simulink library "did"  (R2021b)
settings: Solver=VariableStepAuto  StartTime=0.0  StopTime=10.0  RelTol=1e-3
undefined symbols (not defined in the file or in its folder): ADID_DODRange_pct, ADID_SOCRange_pct, ADID_TempRange_C, DiscIntNeverNeededParam, ENUM_CHRGPLUGSTA_AC, ENUM_CHRGPLUGSTA_DC, ENUM_CHRGPLUGSTA_NONE, ENUM_DRIVETRAIN_AWD, ENUM_DRIVETRAIN_FWD, ENUM_DRIVETRAIN_RWD, ENUM_EXTCHRGSTS_CHARGING, ENUM_OBCV2LSTA_WORKING, ENUM_PWRSTASW_READY, ENUM_VEHICLETYPE_D31HAWD, ENUM_VEHICLETYPE_D31HRWD, HOUR2SEC, HUNDRED, KDID_CPSAVehSpdThres_kph, KDID_DIDModelVersion_raw, KDID_DoDChrgCycle_s, KDID_FiveKmEquivEnergy_Wh, KDID_FlashInitDIDModelVersion_raw, KDID_IPSAVehSpdThres_kph, KDID_PropActiveTripThres_s, KDID_PSARResetThres_sec, KDID_RESSCNTSDODRNGAXIS_enum, KDID_RESSTIMESOCRNGAXIS_enum, KDID_RESSTTEMPRNGAXIS_enum, KDID_WarnUpPropActiveThres_s, KDID_WarnUpVehOperIdleThres_mph, KDID_WarnUpVehOperIdleThres_s, KDID_WarnUpVehOperThres_mph, KDID_WarnUpVehOperThres_s, KPH2MPH, KXX2XX, MINUSONE_FLOAT, ONE_FLOAT, ONE_INT, ONE_INT16, ONE_PERCENT, TRUE, UINT16_MAX, UINT32_MAX, XX2KXX, ZERO_FLOAT, ZERO_INT, ZERO_INT16, ZERO_INT32
libraries: hcu_lib x112, simulink x10, nmm x1
(part 2 of 4)

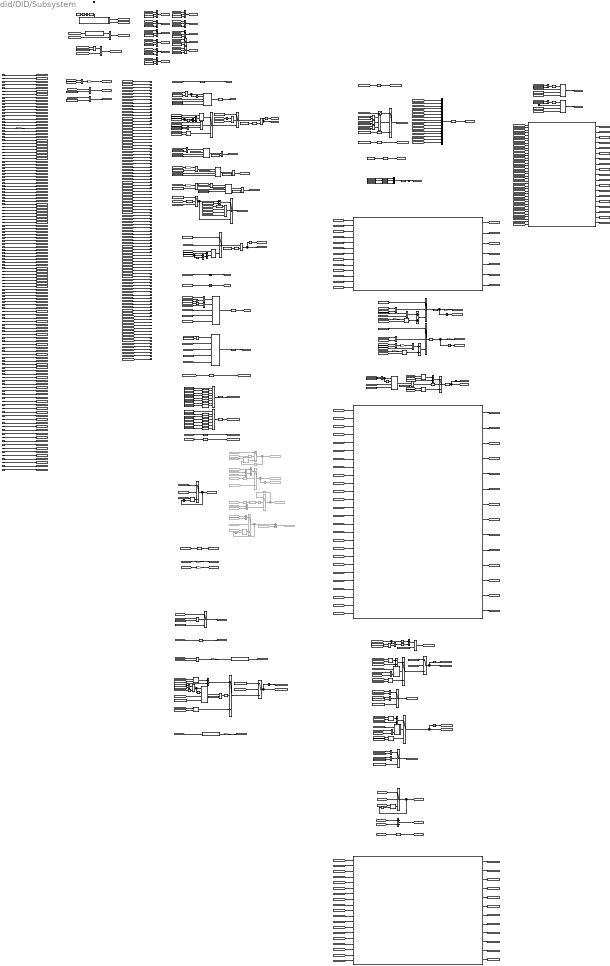
== system did/DID/Subsystem ==
  note: Flash data selector
  note: Model Version
  note: 0xF810: Protocol Identification
  note: 0xF896: Total Number of Propulsion System Active Events
  note: code_clear ??
  note: 0xF44D: Engine run time while MIL activated
  note: 0xF431: Distance traveled since DTCs cleared
  note: 0xF430: Number of warm-ups since DTCs cleared
  note: add debounce?
  note: 0xF421: Distance Traveled While MIL is Activated
  note: 0xF41F: Time Since Engine Start
  note: 0xF40D: Vehicle Speed Sensor
  note: 0xF449: Accelerator Pedal Position D
  note: 0xF44A: Accelerator Pedal Position E
  note: add debounce?
  note: 0xF44E: Engine run time since DTCs cleared
  note: 0xF45B: Hybrid Battery Pack Remaining Charge
  note: 0xF49A: Hybrid/EV Battery System Voltage
  note: 0xF4D1
  note: 0xF4DA
  note: 0xF4D4
  note: 0xF4B9
  note: 0xF4D6
  note: 0xF4D0
  note: SOH?
  note: 0xF4A6
  note: 0xF4B2
  note: Annex G
  note: Annex B
  note: 0xF802: Vehicle Identification Number
  note: 0xF804: Calibration Identifications
  note: 0xF813: Certification Test Group/Engine Family Number
  note: 0xF80A: ECUNAME
  note: 0xF881: High Voltage Battery Net Amp Hours
  note: 0xF882: Ignition Counter
  note: 0xF88C: Positive Kinetic Energy
  note: 0xF88D: Total Distance Travelled
  task_time_s : Inport
  VTQD_VehActSpd_kph : Inport  Port=2
  VPMM_SysPowerMode_enum : Inport  Port=3
  VPMM_DrivetrainSelect_enum : Inport  Port=4
  VDDM_VehMalfunLevel_enum : Inport  Port=5
  VDDM_LimpHomeActTmp_flg : Inport  Port=6
  VDDM_EnterNewOperCyc_flg : Inport  Port=7
  VINP_CANMsgValidESC1_flg : Inport  Port=8
  VINP_ODOMETER_km : Inport  Port=9
  VINP_CANMsgValidMETER1_flg : Inport  Port=10
  VINP_ClearDTCcmd_flg : Inport  Port=11
  VDHP_LowIdleAccPedal_flg : Inport  Port=12
  VDHP_EAPS1NRM_pct : Inport  Port=13
  VDHP_EAPS2NRM_pct : Inport  Port=14
  VINP_HVBattSOC_pct : Inport  Port=15
  VINP_HVBattPackVolt_V : Inport  Port=16
  VINP_ExtChrgSta_enum : Inport  Port=17
  VINP_HVBattCurr_A : Inport  Port=18
  VINP_HVBattVolt_V : Inport  Port=19
  VINP_ChrgPlugSta_enum : Inport  Port=20
  VINP_HVBPwrAvailChrg_kW : Inport  Port=21
  VINP_HVBCellVoltMax_mV : Inport  Port=22
  VINP_HVBCellVoltMin_mV : Inport  Port=23
  VINP_HVBSOH_pct : Inport  Port=24
  VINP_CANMsgValidMCUBR1_flg : Inport  Port=25
  VINP_CANMsgValidBMS6_flg : Inport  Port=26
  VINP_CANMsgValidBMS1_flg : Inport  Port=27
  VINP_CANMsgValidCCU2_flg : Inport  Port=28
  VINP_CANMsgValidBMS4_flg : Inport  Port=29
  VINP_CellTempAvg_C : Inport  Port=30
  VINP_OBCV2LSta_enum : Inport  Port=31
  VINP_RrMCUDCBusCurr_A : Inport  Port=32
  VINP_RrMCUDCBusVolt_V : Inport  Port=33
  VINP_FrMCUDCBusCurr_A : Inport  Port=34
  VINP_FrMCUDCBusVolt_V : Inport  Port=35
  VINP_CANMsgValidMCUBF1_flg : Inport  Port=36
  VINP_HVBMTempMax_C : Inport  Port=37
  VINP_HVBMTempMin_C : Inport  Port=38
  VINP_MCUBRRealPwrKwSta_kW : Inport  Port=39
  VINP_MCUBFRealPwrKwSta_kW : Inport  Port=40
  VINP_CANMsgValidBMS3_flg : Inport  Port=41
  VINP_VehicleType_enum : Inport  Port=42
  VINP_CarModel1_cnt : Inport  Port=43
  VINP_CarModel2_cnt : Inport  Port=44
  VINP_CarModel3_cnt : Inport  Port=45
  VINP_ECU1_cnt : Inport  Port=46
  VINP_ECU2_cnt : Inport  Port=47
  VINP_Major1_cnt : Inport  Port=48
  VINP_Major2_cnt : Inport  Port=49
  VINP_Minor1_cnt : Inport  Port=50
  VINP_Minor2_cnt : Inport  Port=51
  VINP_Patch1_cnt : Inport  Port=52
  VINP_Patch2_cnt : Inport  Port=53
  VINP_Country1_cnt : Inport  Port=54
  VINP_Country2_cnt : Inport  Port=55
  VINP_Variation_cnt : Inport  Port=56
  VINP_ECUGen1_cnt : Inport  Port=57
  VINP_ECUGen2_cnt : Inport  Port=58
  VINP_FlashMILDIST_km : Inport  Port=59
  VINP_FlashWARMUPS_cnt : Inport  Port=60
  VINP_FlashDelayCLRDIST_km : Inport  Port=61
  VINP_FlashMILTime_min : Inport  Port=62
  VINP_FlashCLRTime_min : Inport  Port=63
  VINP_FlashNUMPSATRIPSFLTMEMCLR_cnt : Inport  Port=64
  VINP_FlashPSAR_sec : Inport  Port=65
  VINP_FlashPSAL_sec : Inport  Port=66
  VINP_FlashIPSAR_sec : Inport  Port=67
  VINP_FlashIPSAL_sec : Inport  Port=68
  VINP_FlashCPSAR_sec : Inport  Port=69
  VINP_FlashCPSAL_sec : Inport  Port=70
  VINP_FlashHVBNAH_Ah : Inport  Port=71
  VINP_FlashIGNCNTR_cnt : Inport  Port=72
  VINP_FlashTNBCPSAR_Ahr : Inport  Port=73
  VINP_FlashTNBCPSAL_Ahr : Inport  Port=74
  VINP_FlashTNECPSAR_kWh : Inport  Port=75
  VINP_FlashTNECPSAL_kWh : Inport  Port=76
  VINP_FlashTEBPSAR_kWh : Inport  Port=77
  VINP_FlashTEBPSAL_kWh : Inport  Port=78
  VINP_FlashTGEOVCR_kWh : Inport  Port=79
  VINP_FlashTGEOVCL_kWh : Inport  Port=80
  VINP_FlashGECHGOVCDCR_kWh : Inport  Port=81
  VINP_FlashGECHGOVCDCL_kWh : Inport  Port=82
  VINP_FlashGECHGOVCACR_kWh : Inport  Port=83
  VINP_FlashGECHGOVCACL_kWh : Inport  Port=84
  VINP_FlashRESSV2XENNONPSAR_kWh : Inport  Port=85
  VINP_FlashRESSV2XENNONPSAL_kWh : Inport  Port=86
  VINP_FlashODOMETER_km : Inport  Port=87
  VINP_FlashPKERNumerator_kphsqr : Inport  Port=88
  VINP_FlashPKELNumerator_kphsqr : Inport  Port=89
  VINP_FlashResetCDEODTR_km : Inport  Port=90
  VINP_FlashTempPSAR_sec : Inport  Port=91
  VINP_FlashAvgBattTempPSAR_C : Inport  Port=92
  VINP_FlashTempPSAL_sec : Inport  Port=93
  VINP_FlashAvgBattTempPSAL_C : Inport  Port=94
  VINP_FlashOVCR_sec : Inport  Port=95
  VINP_FlashAvgBattTempOVCR_C : Inport  Port=96
  VINP_FlashOVCL_sec : Inport  Port=97
  VINP_FlashAvgBattTempOVCL_C : Inport  Port=98
  VINP_FlashOFFR_sec : Inport  Port=99
  VINP_FlashAvgBattTempOFFR_C : Inport  Port=100
  VINP_FlashOFFL_sec : Inport  Port=101
  VINP_FlashAvgBattTempOFFL_C : Inport  Port=102
  VINP_FlashHVBNE_kWh : Inport  Port=103
  VINP_FlashQTYPSATRIPSR_cnt : Inport  Port=104
  VINP_FlashQTYPSATRIPSL_cnt : Inport  Port=105
  VINP_FlashRESSCNTDODRNGR_cnt : Inport  Port=106
  VINP_FlashETMBTOER_kWh : Inport  Port=107
  VINP_FlashETMBTOEL_kWh : Inport  Port=108
  VINP_FlashRESSCNTDODRNGL_cnt : Inport  Port=109
  VINP_FlashETMATOER_kWh : Inport  Port=110
  VINP_FlashETMATOEL_kWh : Inport  Port=111
  VINP_FlashRESSTIMESOCPSARNGR_s : Inport  Port=112
  VINP_FlashRESSTIMESOCPSARNGL_s : Inport  Port=113
  VINP_FlashRESSTIMESOCCHGRNGR_s : Inport  Port=114
  VINP_FlashRESSTIMESOCOFFRNGL_s : Inport  Port=115
  VINP_FlashMAXBATTEMPL_C : Inport  Port=116
  VINP_FlashMINBATTEMPL_C : Inport  Port=117
  VINP_FlashRESSTIMESOCCHGRNGL_s : Inport  Port=118
  VINP_FlashRESSTIMESOCOFFRNGR_s : Inport  Port=119
  VINP_FlashAVGBATTEMPL_sec : Inport  Port=120
  VINP_FlashAVGBATTEMPL_C : Inport  Port=121
  VINP_VinCode_cnt : Inport  Port=122
  VINP_FlashModelVersion_raw : Inport  Port=123
  VINP_FlashModelVersionChksum_raw : Inport  Port=124
  Enable : EnablePort
  0xF819: Total Propulsion System Active Time : Subsystem
  0xF885 - 0xF88B : Subsystem
  0xF88E - 0xF890 : Subsystem
  0xF898-0xF8 : Subsystem
  1-D Lookup Table : Lookup_n-D  NumberOfTableDimensions=1  BreakpointsForDimension1=[ENUM_DRIVETRAIN_RWD;ENUM_DRIVETRAIN_FWD;ENUM_DRIVETRAIN_AWD]  Table=[uint8('R');uint8('F');uint8('A')]  InterpMethod=Nearest  InternalRulePriority=Speed  RndMeth=Simplest  InputSameDT=on
  AND : Logic  AllPortsSameDT=off  OutDataTypeStr=boolean
  AND2 : Logic  AllPortsSameDT=off  OutDataTypeStr=boolean
  AND6 : Logic  AllPortsSameDT=off  OutDataTypeStr=boolean
  Add{,1..3,6} (5 alike) : Sum
  Bitwise OR1 : simulink/Logic and Bit Operations/Bitwise Operator  logicop=OR  UseBitMask=off  NumInputPorts=7  BitMask=bin2dec('00000000000000000000')  BitMaskRealWorld=Stored Integer
  Bitwise OR123 : simulink/Logic and Bit Operations/Bitwise Operator  logicop=OR  UseBitMask=off  NumInputPorts=8  BitMask=bin2dec('00000000000000000000')  BitMaskRealWorld=Stored Integer
  Cast To Boolean : DataTypeConversion  OutDataTypeStr=boolean
  Checksum : Subsystem
  Constant{,5..6,18..19,25..26,28,34} (9 alike) : Constant  Value=ENUM_PWRSTASW_READY
  Constant1 : Constant  Value=UINT32_MAX
  Constant10 : Constant  Value=KDID_WarnUpVehOperThres_s
  Constant{3,16,32,59,65..68,105,113} (10 alike) : Constant  Value=ZERO_FLOAT
  Constant11 : Constant  Value=KDID_WarnUpVehOperThres_s
  Constant12 : Constant  Value=KDID_WarnUpVehOperIdleThres_s
  Constant13 : Constant  Value=KDID_WarnUpVehOperIdleThres_s
  Constant14 : Constant  Value=KDID_WarnUpVehOperIdleThres_mph
  Constant{15,42,44..45,47..48,51..54,57..58,61..63,69..77} (24 alike) : Constant  Value=ZERO_INT
  Constant{4,17,20,24} (4 alike) : Constant  Value=UINT16_MAX
  Constant2 : Constant  Value=ONE_INT
  Constant21 : Constant  Value=ZERO_INT32
  Constant22 : Constant  Value=ONE_PERCENT  OutDataTypeStr=single
  Constant23 : Constant  Value=ZERO_INT16
  Constant27 : Constant  Value=ONE_INT16
  Constant{29..30,38,49} (4 alike) : Constant  Value=KDID_PropActiveTripThres_s
  Constant31 : Constant  Value=ENUM_EXTCHRGSTS_CHARGING
  Constant33 : Constant  Value=UINT32_MAX
  Constant35 : Constant  Value=UINT32_MAX
  Constant36 : Constant  Value=ONE_INT
  Constant37 : Constant  Value=ZERO_FLOAT  OutDataTypeStr=uint16
  Constant39 : Constant  Value=ENUM_DRIVETRAIN_RWD
  Constant40 : Constant  Value=ENUM_DRIVETRAIN_RWD
  Constant41 : Constant  Value=ENUM_DRIVETRAIN_RWD
  Constant43 : Constant  Value=ONE_INT
  Constant46 : Constant  Value=ONE_PERCENT  OutDataTypeStr=single
  Constant50 : Constant  Value=ZERO_FLOAT  OutDataTypeStr=single
  Constant55 : Constant  Value=KDID_FlashInitDIDModelVersion_raw
  Constant56 : Constant  Value=ZERO_FLOAT  OutDataTypeStr=single
  Constant60 : Constant  Value=ONE_FLOAT
  Constant64 : Constant  Value=TRUE
  Constant7 : Constant  Value=KDID_WarnUpPropActiveThres_s
  Constant79 : Constant  Value=ONE_INT16
  Constant8 : Constant  Value=KDID_WarnUpPropActiveThres_s
  Constant9 : Constant  Value=KDID_WarnUpVehOperThres_mph
  Data Type Conversion{,2..3,23,25} (5 alike) : DataTypeConversion  OutDataTypeStr=single
  Data Type Conversion{1,9..10,29} (4 alike) : DataTypeConversion  OutDataTypeStr=uint16
  Data Type Conversion{4..5,11,14,16..17} (6 alike) : DataTypeConversion  OutDataTypeStr=uint8
  Data Type Conversion{6..8,12..13,15} (6 alike) : DataTypeConversion
  Delay : Delay  DelayLengthSource=Input port  DelayLengthUpperLimit=255
      settings: InputPortMap=u0,p1
  Delay1 : Delay
  Delay2 : Delay  Commented=on  DelayLength=1
  Detect Decrease : simulink/Logic and Bit Operations/Detect Decrease  Commented=on  vinit=0.0  OutDataTypeStr=boolean
  Detect Increase{,1..3} (4 alike) : simulink/Logic and Bit Operations/Detect Increase  vinit=0.0  OutDataTypeStr=boolean
  Detect Increase4 : simulink/Logic and Bit Operations/Detect Increase  Commented=on  vinit=0.0  OutDataTypeStr=boolean
  Detect Increase5 : simulink/Logic and Bit Operations/Detect Increase  Commented=on  vinit=0.0  OutDataTypeStr=boolean
  Divide : Product  Inputs=*/
  Divide1 : Product  Inputs=*/
  Divide2 : Product  Inputs=*/
  Equal{,1..2,8..10,12..13,15..18,21..22} (14 alike) : RelationalOperator  Operator===  OutDataTypeStr=boolean  RndMeth=Simplest
  Equal{3..5,7,11,14,23} (7 alike) : RelationalOperator  OutDataTypeStr=boolean  RndMeth=Simplest
  Equal19 : RelationalOperator  Operator=>  OutDataTypeStr=boolean  RndMeth=Simplest
  Equal20 : RelationalOperator  Operator=>  OutDataTypeStr=boolean  RndMeth=Simplest
  Equal6 : RelationalOperator  Operator=<=  OutDataTypeStr=boolean  RndMeth=Simplest
  From{357,368,371,373,381} (5 alike) : From  Commented=on  GotoTag=VINP_ODOMETER_km
  From367 : From  Commented=on  GotoTag=VINP_FlashODOMETER_km
  From369 : From  Commented=on  GotoTag=VINP_FlashODOMETER_km
  From{370,375,379..380} (4 alike) : From  Commented=on  GotoTag=VINP_CANMsgValidMETER1_flg
  From372 : From  Commented=on  GotoTag=VDID_ODOMETERLostConn_km
  From374 : From  Commented=on  GotoTag=VDID_ODOMETERLostDelay_km
  From376 : From  Commented=on  GotoTag=VDID_ODOMETERLostDelay_km
  From377 : From  Commented=on  GotoTag=VDID_ODOMETERLost_km
  From378 : From  Commented=on  GotoTag=VINP_FlashODOMETERLost_km
  Gain : Gain  Gain=KPH2MPH
  Gain1 : Gain  Gain=KPH2MPH
  Gain{2..3,14,20} (4 alike) : Gain  Gain=1/HOUR2SEC
  Gain19 : Gain  Gain=MINUSONE_FLOAT
  Gain21 : Gain  Gain=HOUR2SEC
  Gain{5..6,8,27} (4 alike) : Gain  Gain=XX2KXX
  Gain7 : Gain  Gain=HOUR2SEC
  Goto247 : Goto  Commented=on  GotoTag=VDID_ODOMETERLostConn_km
  Goto248 : Goto  Commented=on  GotoTag=VDID_ODOMETERLost_km
  Goto249 : Goto  Commented=on  GotoTag=VDID_ODOMETERLostDelay_km
  Goto250 : Goto  Commented=on  GotoTag=VDID_ODOMETER_km
  Goto251 : Goto  Commented=on  GotoTag=VINP_FlashODOMETERLost_km
  Ground : Ground
  Initial Value{,1..8,11..12,34..37} (15 alike) : hcu_lib/Basic_Blocks/Initial Value
  Initial Value10 : hcu_lib/Basic_Blocks/Initial Value  Commented=on
  Initial Value9 : hcu_lib/Basic_Blocks/Initial Value  Commented=on
  Initializable_U32counter : hcu_lib/Basic_Blocks/Initializable_U32counter
  Initializable_U32counter1 : hcu_lib/Basic_Blocks/Initializable_U32counter
  Latch : hcu_lib/Basic_Blocks/Latch
  Latch1 : hcu_lib/Basic_Blocks/Latch
  Latch2 : hcu_lib/Basic_Blocks/Latch  Commented=on
  Logical Operator{,5..7} (4 alike) : Logic  Operator=OR  AllPortsSameDT=off  OutDataTypeStr=boolean
  Logical Operator1 : Logic  Inputs=3  AllPortsSameDT=off  OutDataTypeStr=boolean
  Logical Operator2 : Logic  Inputs=4  AllPortsSameDT=off  OutDataTypeStr=boolean
  Logical Operator3 : Logic  AllPortsSameDT=off  OutDataTypeStr=boolean
  Logical Operator4 : Logic  AllPortsSameDT=off  OutDataTypeStr=boolean
  Logical Operator8 : Logic  Operator=NOT  AllPortsSameDT=off  OutDataTypeStr=boolean
  Logical Operator9 : Logic  AllPortsSameDT=off  OutDataTypeStr=boolean
  Max : MinMax  Inputs=2
  Max1 : MinMax  Inputs=2
  Max3 : MinMax  Function=max  Inputs=2
  Min14 : MinMax  Function=max  Inputs=2
  Min15 : MinMax  Inputs=2
  Minus : Sum  Inputs=+-
  Minus1 : Sum
  Minus2 : Sum
  Minus{3..6} (4 alike) : Sum  Commented=on  Inputs=+-
  Minus7 : Sum  Commented=on
  Minutes_Counter : hcu_lib/Basic_Blocks/Minutes_Counter
  Minutes_Counter1 : hcu_lib/Basic_Blocks/Minutes_Counter
  Mux : Mux  Inputs=3
  Mux1 : Mux  Inputs=16
  NOT{,1..4,6} (6 alike) : Logic  Operator=NOT  AllPortsSameDT=off  OutDataTypeStr=boolean
  OR : Logic  Operator=OR  Inputs=3  AllPortsSameDT=off  OutDataTypeStr=boolean
  Product{,1..2,4,27} (5 alike) : Product
  Reshape : Reshape
  Riemann Integral : hcu_lib/Basic_Blocks/Riemann Integral  Ts=0.005  Total_T=1
  Riemann Integral1 : hcu_lib/Basic_Blocks/Riemann Integral  Ts=0.005  Total_T=1
  Saturation : Saturate  UpperLimit=HUNDRED  LowerLimit=ZERO_FLOAT  OutDataTypeStr=single
  Saturation1 : Saturate  UpperLimit=HUNDRED  LowerLimit=ZERO_FLOAT  OutDataTypeStr=single
  Scheduler : Stateflow chart  TreatAsAtomicUnit=on
  Scheduler1 : Stateflow chart  TreatAsAtomicUnit=on
  Seconds_Counter : hcu_lib/Basic_Blocks/Seconds_Counter
  Shift Arithmetic1 : ArithShift  BitShiftNumber=4  BitShiftDirection=Left
  Shift Arithmetic10 : ArithShift  BitShiftNumber=3  BitShiftDirection=Left
  Shift Arithmetic11 : ArithShift  BitShiftNumber=7  BitShiftDirection=Left
  Shift Arithmetic2 : ArithShift  BitShiftNumber=5  BitShiftDirection=Left
  Shift Arithmetic3 : ArithShift  BitShiftNumber=6  BitShiftDirection=Left
  Shift Arithmetic311 : ArithShift  BitShiftNumber=1  BitShiftDirection=Left
  Shift Arithmetic312 : ArithShift  BitShiftNumber=2  BitShiftDirection=Left
  Shift Arithmetic313 : ArithShift  BitShiftNumber=3  BitShiftDirection=Left
  Shift Arithmetic4 : ArithShift  BitShiftNumber=7  BitShiftDirection=Left
  Shift Arithmetic5 : ArithShift  BitShiftNumber=4  BitShiftDirection=Left
  Shift Arithmetic6 : ArithShift  BitShiftNumber=5  BitShiftDirection=Left
  Shift Arithmetic7 : ArithShift  BitShiftNumber=6  BitShiftDirection=Left
  Shift Arithmetic8 : ArithShift  BitShiftNumber=1  BitShiftDirection=Left
  Square : Math  Operator=square  SaturateOnIntegerOverflow=on
  Square1 : Math  Operator=square  SaturateOnIntegerOverflow=on
  String Constant : StringConstant  String="\"EVCM\""
  String Constant1 : StringConstant  String="\"-\""
  String Constant2 : StringConstant  String="\"ElecVehicleCtrl\""
  String Constant3 : StringConstant  String="\"0\""
  String Constant4 : StringConstant  String="\"S\""
  String to ASCII : StringToASCII  OutputVectorSize=4
  String to ASCII1 : StringToASCII  OutputVectorSize=1
  String to ASCII2 : StringToASCII  OutputVectorSize=15
  String to ASCII3 : StringToASCII  OutputVectorSize=1
  String to ASCII4 : StringToASCII  OutputVectorSize=1
  Subsystem : Subsystem
  Subtract : Sum  Inputs=+-
  Subtract1 : Sum  Inputs=+-
  Subtract2 : Sum
  Subtract3 : Sum
  Subtract6 : Sum  Inputs=+-
  Switch{,1..9,11,13..27,61} (27 alike) : Switch  Criteria=u2 > Threshold
  Switch10 : Switch  Criteria=u2 ~= 0
      settings: AttributesFormatString=<%<Criteria>>
  Switch12 : Switch  Criteria=u2 ~= 0
      settings: AttributesFormatString=<%<Criteria>>
  Switch{28..31} (4 alike) : Switch  Commented=on  Criteria=u2 > Threshold
  Switch60 : Switch  Criteria=u2 ~= 0
      settings: AttributesFormatString=<%<Criteria>>
  Timer{1..3,5..6} (5 alike) : hcu_lib/Basic_Blocks/Timer
  Unit Delay{,1..2,4..7,11,13..14,20,23} (12 alike) : UnitDelay  SampleTime=-1  HasFrameUpgradeWarning=on
  Unit Delay{3,8..10} (4 alike) : UnitDelay  Commented=on  SampleTime=-1  HasFrameUpgradeWarning=on
  VDID_VSS_kph : Outport
  VDID_RUNTM_s : Outport  Port=2
  VDID_MILDIST_km : Outport  Port=3
  VDID_WARMUPS_cnt : Outport  Port=4
  VDID_CLRDIST_km : Outport  Port=5
  VDID_APPD_pct : Outport  Port=6
  VDID_APPE_pct : Outport  Port=7
  VDID_MILTIME_min : Outport  Port=8
  VDID_CLRTIME_min : Outport  Port=9
  VDID_BATSOC_pct : Outport  Port=10
  VDID_HEVBATT_V : Outport  Port=11
  VDID_ODOMETER_km : Outport  Port=12
  VDID_BATSOH_pct : Outport  Port=13
  VDID_HVBCellVoltMin_V : Outport  Port=14
  VDID_HVBCellVoltMax_V : Outport  Port=15
  VDID_HVESSCHARGELIM_kW : Outport  Port=16
  VDID_HVESSCHARGEACT_kW : Outport  Port=17
  VDID_HVESSENER_Whps : Outport  Port=18
  VDID_NUMPSATRIPSFLTMEMCLR_cnt : Outport  Port=19
  VDID_HVBattCurr_Ahps : Outport  Port=20
  VDID_PSAR_sec : Outport  Port=21
  VDID_PSAL_sec : Outport  Port=22
  VDID_IPSAR_sec : Outport  Port=23
  VDID_IPSAL_sec : Outport  Port=24
  VDID_CPSAR_sec : Outport  Port=25
  VDID_CPSAL_sec : Outport  Port=26
  VDID_HVBNAH_Ahr : Outport  Port=27
  VDID_HVBNE_kWh : Outport  Port=28
  VDID_IGNCNTR_cnt : Outport  Port=29
  VDID_TNBCPSAR_Ahr : Outport  Port=30
  VDID_TNBCPSAL_Ahr : Outport  Port=31
  VDID_TNECPSAR_kWh : Outport  Port=32
  VDID_TNECPSAL_kWh : Outport  Port=33
  VDID_TEBPSAR_kWh : Outport  Port=34
  VDID_TEBPSAL_kWh : Outport  Port=35
  VDID_TGEOVCR_kWh : Outport  Port=36
  VDID_TGEOVCL_kWh : Outport  Port=37
  VDID_GECHGOVCDCR_kWh : Outport  Port=38
  VDID_GECHGOVCDCL_kWh : Outport  Port=39
  VDID_GECHGOVCACR_kWh : Outport  Port=40
  VDID_GECHGOVCACL_kWh : Outport  Port=41
  VDID_RESSV2XENNONPSAR_kWh : Outport  Port=42
  VDID_RESSV2XENNONPSAL_kWh : Outport  Port=43
  VDID_PKER_kphsqr : Outport  Port=44
  VDID_PKEL_kphsqr : Outport  Port=45
  VDID_ResetCDEODTR_km : Outport  Port=46
  VDID_CDEODTR_km : Outport  Port=47
  VDID_CDEODTL_km : Outport  Port=48
  VDID_AvgBattTempPSAR_C : Outport  Port=49
  VDID_AvgBattTempPSAL_C : Outport  Port=50
  VDID_AvgBattTempOVCR_C : Outport  Port=51
  VDID_AvgBattTempOVCL_C : Outport  Port=52
  VDID_AvgBattTempOFFR_C : Outport  Port=53
  VDID_AvgBattTempOFFL_C : Outport  Port=54
  VDID_QTYPSATRIPSR_cnt : Outport  Port=55
  VDID_QTYPSATRIPSL_cnt : Outport  Port=56
  VDID_RESSCNTDODRNGR_cnt : Outport  Port=57
  VDID_RESSCNTDODRNGL_cnt : Outport  Port=58
  VDID_ETMATOER_kWh : Outport  Port=59
  VDID_ETMATOEL_kWh : Outport  Port=60
  VDID_ETMBTOER_kWh : Outport  Port=61
  VDID_ETMBTOEL_kWh : Outport  Port=62
  VDID_RESSTIMESOCPSARNGR_s : Outport  Port=63
  VDID_RESSTIMESOCPSARNGL_s : Outport  Port=64
  VDID_RESSTIMESOCCHGRNGR_s : Outport  Port=65
  VDID_RESSTIMESOCCHGRNGL_s : Outport  Port=66
  VDID_RESSTIMESOCOFFRNGR_s : Outport  Port=67
  VDID_RESSTIMESOCOFFRNGL_s : Outport  Port=68
  VDID_MAXBATTEMPL_C : Outport  Port=69
  VDID_MINBATTEMPL_C : Outport  Port=70
  VDID_AVGBATTEMPL_C : Outport  Port=71
  VDID_PRO TOCOLID_enum : Outport  Port=72
  VDID_RESSTTEMPRNGAXIS_enum : Outport  Port=73
  VDID_RESSTIMESOCRNGAXIS_enum : Outport  Port=74
  VDID_RESSCNTSDODRNGAXIS_enum : Outport  Port=75
  VDID_CALID_cnt : Outport  Port=76
  VDID_ECUNAME_cnt : Outport  Port=77
  VDID_PKERNumerator_kphsqr : Outport  Port=78
  VDID_PKELNumerator_kphsqr : Outport  Port=79
  VDID_BattTempPSAR_sec : Outport  Port=80
  VDID_BattTempPSAL_sec : Outport  Port=81
  VDID_OVCR_sec : Outport  Port=82
  VDID_OVCL_sec : Outport  Port=83
  VDID_OFFR_sec : Outport  Port=84
  VDID_OFFL_sec : Outport  Port=85
  VDID_AVGBATTEMPL_sec : Outport  Port=86
  VDID_VinCode_cnt : Outport  Port=87
  VDID_STASUP_enum : Outport  Port=88
  VDID_HEVMODE_enum : Outport  Port=89
  VDID_HVBATT_A : Outport  Port=90
  VDID_DIDModelVersion_raw : Outport  Port=91
  VDID_DIDModelVersionChksum_raw : Outport  Port=92
  wires:
  task_time_s/1 -> [task_time_s]
  VTQD_VehActSpd_kph/1 -> [VTQD_VehActSpd_kph]
  [VTQD_VehActSpd_kph] -> Data Type Conversion/1
  Data Type Conversion/1 -> [VDID_VSS_kph]
  VPMM_SysPowerMode_enum/1 -> [VPMM_SysPowerMode_enum]
  [VPMM_SysPowerMode_enum] -> Equal/1
  Constant/1 -> Equal/2
  Equal/1 -> NOT1/1, Seconds_Counter/1
  NOT1/1 -> Seconds_Counter/2
  [task_time_s] -> Seconds_Counter/3
  Constant1/1 -> Seconds_Counter/4
  Seconds_Counter/1 -> Data Type Conversion1/1
  Data Type Conversion1/1 -> [VDID_RUNTM_s]
  VDDM_VehMalfunLevel_enum/1 -> [VDDM_VehMalfunLevel_enum]
  VINP_ODOMETER_km/1 -> [VINP_ODOMETER_km]
  Unit Delay1/1 -> Subtract/2
  Subtract/1 -> Add/2
  Unit Delay/1 -> [VDID_DelayMILDIST_km]
  Switch/1 -> Switch1/3
  VINP_ClearDTCcmd_flg/1 -> [VINP_ClearDTCcmd_flg]
  [VDDM_LimpHomeActTmp_flg] -> NOT/1
  NOT/1 -> Logical Operator/1
  [VINP_ClearDTCcmd_flg] -> Logical Operator/2
  Constant3/1 -> Switch1/1
  Switch1/1 -> Max/1
  Max/1 -> Unit Delay/1, [VDID_MILDIST_km]
  VINP_CANMsgValidMETER1_flg/1 -> [VINP_CANMsgValidMETER1_flg]
  [VDDM_LimpHomeActTmp_flg] -> Logical Operator1/1
  Logical Operator1/1 -> Switch/2
  [VDID_ODOMETER_km] -> Unit Delay1/1, Subtract/1
  Constant5/1 -> Equal2/2
  [VPMM_SysPowerMode_enum] -> Equal2/1
  Equal2/1 -> Logical Operator1/3
  VDDM_LimpHomeActTmp_flg/1 -> [VDDM_LimpHomeActTmp_flg]
  Logical Operator/1 -> Switch1/2
  VDDM_EnterNewOperCyc_flg/1 -> [VDDM_EnterNewOperCyc_flg]
  [VDDM_EnterNewOperCyc_flg] -> Latch/1
  Latch/1 -> Logical Operator2/1
  Switch3/1 -> Add1/1, Switch2/3
  Constant2/1 -> Add1/2
  Add1/1 -> Switch2/1
  Constant6/1 -> Equal1/2
  Constant7/1 -> Timer1/4
  Equal1/1 -> Timer1/1
  [task_time_s] -> Timer1/3
  [VPMM_SysPowerMode_enum] -> Equal1/1
  Timer1/1 -> Equal3/1
  Constant8/1 -> Equal3/2
  [VTQD_VehActSpd_kph] -> Gain/1
  Gain/1 -> Equal4/1
  Constant9/1 -> Equal4/2
  Equal4/1 -> Timer2/1
  [task_time_s] -> Timer2/3
  Constant10/1 -> Timer2/4
  Constant11/1 -> Equal5/2
  Timer2/1 -> Equal5/1
  VDHP_LowIdleAccPedal_flg/1 -> [VDHP_LowIdleAccPedal_flg]
  Timer3/1 -> Equal7/1
  Constant13/1 -> Equal7/2
  Constant12/1 -> Timer3/4
  [task_time_s] -> Timer3/3
  [VINP_ClearDTCcmd_flg] -> Timer3/2
  Constant14/1 -> Equal6/2
  Gain1/1 -> Equal6/1
  [VTQD_VehActSpd_kph] -> Gain1/1
  [VDHP_LowIdleAccPedal_flg] -> AND/1
  AND/1 -> Timer3/1
  Equal6/1 -> AND/2
  Equal3/1 -> [KDID_WarnUpPropActive_flg]
  Equal5/1 -> [KDID_WarnUpVehOper_flg]
  Equal7/1 -> [KDID_WarnUpVehOperIdle_flg]
  [KDID_WarnUpPropActive_flg] -> Logical Operator2/2
  [KDID_WarnUpVehOper_flg] -> Logical Operator2/3
  [KDID_WarnUpVehOperIdle_flg] -> Logical Operator2/4
  Logical Operator2/1 -> Switch2/2
  [VINP_FlashWARMUPS_cnt] -> Switch3/3
  [VINP_ClearDTCcmd_flg] -> Latch1/1
  Constant15/1 -> Switch3/1
  Switch2/1 -> [VDID_WARMUPS_cnt]
  Latch1/1 -> Switch3/2
  [VINP_ClearDTCcmd_flg] -> Switch4/2
  [VDID_ODOMETER_km] -> Unit Delay2/1, Subtract1/1
  Unit Delay2/1 -> Subtract1/2
  Constant16/1 -> Switch4/1
  Switch4/1 -> Max1/1
  Unit Delay4/1 -> [VDID_DelayCLRDIST_km]
  VDHP_EAPS1NRM_pct/1 -> [VDHP_EAPS1NRM_pct]
  VDHP_EAPS2NRM_pct/1 -> [VDHP_EAPS2NRM_pct]
  [VDHP_EAPS1NRM_pct] -> Saturation/1
  [VDHP_EAPS2NRM_pct] -> Saturation1/1
  Saturation1/1 -> [VDID_APPE_pct]
  [VPMM_SysPowerMode_enum] -> Equal8/1
  Constant19/1 -> Equal8/2
  Equal8/1 -> Logical Operator3/2
  [VDDM_LimpHomeActTmp_flg] -> Logical Operator3/1
  [VDDM_LimpHomeActTmp_flg] -> NOT2/1
  [VINP_ClearDTCcmd_flg] -> Timer2/2
  [VINP_ClearDTCcmd_flg] -> Timer1/2
  VINP_HVBattSOC_pct/1 -> [VINP_HVBattSOC_pct]
  [VINP_HVBattSOC_pct] -> Data Type Conversion6/1
  Data Type Conversion6/1 -> [VDID_BATSOC_pct]  "VDID_BATSOC_pct"
  VINP_HVBattPackVolt_V/1 -> [VINP_HVBattPackVolt_V]
  [VINP_HVBattVolt_V] -> Data Type Conversion7/1
  [VINP_ODOMETER_km] -> Switch9/1
  Gain3/1 -> Riemann Integral1/1
  Switch9/1 -> Unit Delay5/1, [VDID_ODOMETER_km]
  Gain6/1 -> [VDID_HVBCellVoltMax_V]
  [VDID_HVBattPwrChrg_kW] -> Data Type Conversion12/1
  Data Type Conversion8/1 -> [VDID_BATSOH_pct]
  [VINP_HVBSOH_pct] -> Data Type Conversion8/1
  Equal10/1 -> Switch8/2
  [VINP_HVBCellVoltMax_mV] -> Gain6/1
  Switch8/1 -> [VDID_HVESSCHARGELIM_kW]
  [VINP_HVBPwrAvailChrg_kW] -> Switch8/1
  Constant31/1 -> Equal10/2
  [VINP_HVBattVolt_V] -> Product2/2
  Product2/1 -> Gain3/1  "VDID_HVBattPwr_W"
  Riemann Integral1/1 -> [VDID_HVESSENER_Whps]
  Equal11/1 -> Detect Increase/1
  Constant32/1 -> Switch8/3
  Constant29/1 -> Timer6/4
  Detect Increase/1 -> Switch6/2
  [task_time_s] -> Timer6/3
  Timer6/1 -> Equal11/1
  [VINP_ClearDTCcmd_flg] -> Switch5/2
  Gain5/1 -> [VDID_HVBCellVoltMin_V]
  [VINP_HVBCellVoltMin_mV] -> Gain5/1
  [VINP_ExtChrgSta_enum] -> Equal10/1
  Constant30/1 -> Equal11/2
  Constant27/1 -> Add3/2
  Add3/1 -> Switch6/1
  Riemann Integral/1 -> Gain2/1
  Constant23/1 -> Switch5/1
  [VINP_CANMsgValidMETER1_flg] -> Switch9/2
  [VPMM_SysPowerMode_enum] -> Equal9/1
  Constant28/1 -> Equal9/2
  [VDID_DelayMILDIST_km] -> Initial Value1/2
  [VINP_FlashMILDIST_km] -> Initial Value1/1
  Initial Value1/1 -> Switch/3
  [VINP_FlashMILDIST_km] -> Initial Value2/1
  [VDID_DelayMILDIST_km] -> Add/1
  Data Type Conversion9/1 -> [VDID_MILTIME_min]
  Data Type Conversion10/1 -> [VDID_CLRTIME_min]
  Minutes_Counter1/1 -> Data Type Conversion10/1
  Constant18/1 -> Equal12/2
  [VPMM_SysPowerMode_enum] -> Equal12/1
  Equal12/1 -> Minutes_Counter1/1
  Logical Operator3/1 -> Minutes_Counter/1
  [task_time_s] -> Minutes_Counter/3
  Constant20/1 -> Minutes_Counter/4
  Minutes_Counter/1 -> Data Type Conversion9/1
  [task_time_s] -> Minutes_Counter1/3
  Constant24/1 -> Minutes_Counter1/4
  [VINP_ClearDTCcmd_flg] -> Minutes_Counter1/2
  [VDID_HVBattCurr_A] -> Product2/1
  [VINP_ClearDTCcmd_flg] -> NOT3/1
  [VDID_HVBattCurr_A] -> Riemann Integral/1
  Gain2/1 -> [VDID_HVBattCurr_Ahps]
  VINP_ExtChrgSta_enum/1 -> [VINP_ExtChrgSta_enum]
  VINP_HVBattVolt_V/1 -> [VINP_HVBattVolt_V]
  VINP_ChrgPlugSta_enum/1 -> [VINP_ChrgPlugSta_enum]
  VINP_HVBPwrAvailChrg_kW/1 -> [VINP_HVBPwrAvailChrg_kW]
  VINP_HVBCellVoltMax_mV/1 -> [VINP_HVBCellVoltMax_mV]
  VINP_HVBCellVoltMin_mV/1 -> [VINP_HVBCellVoltMin_mV]
  VINP_HVBSOH_pct/1 -> [VINP_HVBSOH_pct]
  VINP_CANMsgValidMCUBR1_flg/1 -> [VINP_CANMsgValidMCUBR1_flg]
  VINP_CANMsgValidESC1_flg/1 -> [VINP_CANMsgValidESC1_flg]
  Switch13/1 -> Data Type Conversion23/1
  Product1/1 -> Minus2/1
  [VINP_DIDResetNetAhrs_flg] -> Logical Operator6/1
  Product/1 -> Minus1/1
  Constant66/1 -> Switch21/1
  Data Type Conversion23/1 -> Gain20/1, Unit Delay13/1
  Switch21/1 -> Data Type Conversion25/1
  Minus2/1 -> Switch21/3
  Constant67/1 -> Switch13/1
  [VINP_DIDResetNetAhrs_flg] -> Logical Operator5/1
  Minus1/1 -> Switch13/3
  [VINP_HVBattVolt_V] -> Product4/2
  [task_time_s] -> Product/2
  [VINP_ClearDTCcmd_flg] -> Logical Operator5/2
  [task_time_s] -> Product1/2
  Logical Operator6/1 -> Switch13/2
  [VINP_ClearDTCcmd_flg] -> Logical Operator6/2
  Logical Operator5/1 -> Switch21/2
  [VDID_HVBattCurr_A] -> Product4/1
  Initial Value11/1 -> Switch22/3
  [VDID_DelayIGNCNTR_cnt] -> Initial Value11/2
  Detect Increase2/1 -> Switch22/2
  [VDID_DelayIGNCNTR_cnt] -> Initial Value12/2
  Unit Delay20/1 -> [VDID_DelayIGNCNTR_cnt]
  [VINP_FlashIGNCNTR_cnt] -> Initial Value11/1
  Switch22/1 -> Data Type Conversion29/1
  Initial Value12/1 -> Add6/1
  Add6/1 -> Switch22/1
  Constant79/1 -> Add6/2
  Data Type Conversion29/1 -> [VDID_IGNCNTR_cnt], Unit Delay20/1
  [VINP_FlashIGNCNTR_cnt] -> Initial Value12/1
  Gain19/1 -> [VDID_HVBattCurr_A]
  Unit Delay13/1 -> [VDID_DelayHVBNAH_As]
  [VDID_FlashHVBNAH_Ah] -> Gain7/1
  [VDID_DelayHVBNAH_As] -> Initial Value7/2
  Initial Value7/1 -> Minus1/2
  [VDID_DelayHVBNE_kWs] -> Initial Value8/2
  [VDID_FlashHVBNE_kWh] -> Gain21/1
  Initial Value8/1 -> Minus2/2
  Unit Delay14/1 -> [VDID_DelayHVBNE_kWs]
  Data Type Conversion25/1 -> Unit Delay14/1, Gain14/1
  Gain21/1 -> Initial Value8/1
  VINP_HVBattCurr_A/1 -> Gain19/1
  [VDID_HVBattCurr_A] -> Product/1
  Gain7/1 -> Initial Value7/1
  Product4/1 -> Gain8/1
  Gain8/1 -> Product1/1  "VDID_HVBattPwr_kW"
  NOT6/1 -> Timer5/2
  Constant25/1 -> Equal18/2
  Equal14/1 -> Detect Increase2/1
  [VPMM_SysPowerMode_enum] -> Equal18/1
  Timer5/1 -> Equal14/1
  Constant49/1 -> Equal14/2
  [task_time_s] -> Timer5/3
  Constant38/1 -> Timer5/4
  Equal18/1 -> NOT6/1, Timer5/1
  [VINP_FlashMILTime_min] -> Minutes_Counter/5
  [VINP_FlashCLRTime_min] -> Minutes_Counter1/5
  Constant105/1 -> Min15/2
  [VDID_HVBattPwr_kW] -> Min15/1
  Min15/1 -> [VDID_HVBattPwrDischrg_kW]
  Min14/1 -> [VDID_HVBattPwrChrg_kW]
  [VDID_HVBattPwr_kW] -> Min14/1
  Constant59/1 -> Min14/2
  Gain27/1 -> [VDID_HVBattPwr_kW]  "VDID_HVBattPwr_kW"
  Product27/1 -> Gain27/1
  [VDID_HVBattCurr_A] -> Product27/1
  [VINP_HVBattVolt_V] -> Product27/2
  Minus/1 -> Max3/1
  Unit Delay23/1 -> [VDID_DelayPKELNumerator_kphsqr]
  [VDID_PKENumeratorOneSec_kphsqr] -> Subtract3/2
  [VINP_FlashPKELNumerator_kphsqr] -> Initial Value37/1
  [VDID_NoteAResetCondition_flg] -> Switch61/2
  [VINP_CANMsgValidMCUBR1_flg] -> AND2/2
  Constant37/1 -> Switch11/3
  Constant113/1 -> Max3/2
  [task_time_s] -> Scheduler1/1(task_time_s)
  [VINP_CANMsgValidESC1_flg] -> AND6/1
  Divide1/1 -> Switch11/1
  Initial Value3/1 -> Switch61/3
  Subtract6/1 -> [VDID_CDEODTR_km]
  [VDID_ResetCDEODTR_km] -> Subtract6/2
  [VDID_ODOMETER_km] -> Data Type Conversion13/1
  [task_time_s] -> Scheduler/1(task_time_s)
  [VDID_ODOMETER_km] -> Subtract6/1
  Scheduler/1(trig_1sec) -> Switch60/2
  Constant22/1 -> Equal19/2
  Switch16/1 -> [VDID_PKEL_kphsqr]
  [VDID_CDEODTR_km] -> Divide1/2
  [VDID_ODOMETER_km] -> Switch61/1
  [VINP_FlashResetCDEODTR_km] -> Initial Value3/1
  Switch61/1 -> Unit Delay6/1, [VDID_ResetCDEODTR_km]
  Switch10/1 -> [VDID_PKERNumerator_kphsqr], Unit Delay11/1
  Switch60/1 -> Switch10/3
  AND2/1 -> Scheduler1/2(trigger)
  [VDID_NoteAResetCondition_flg] -> Switch10/2
  Initial Value36/1 -> Switch12/3
  [VDID_PKELNumerator_kphsqr] -> Divide2/1
  Unit Delay6/1 -> Initial Value3/2
  [VDID_CDEODTL_km] -> Equal20/1
  [task_time_s] -> Divide/2
  [VINP_FlashPKERNumerator_kphsqr] -> Initial Value35/1
  [VDID_PKERNumerator_kphsqr] -> Divide1/1
  Divide2/1 -> Switch16/1
  Delay/1 -> Square1/1
  Initial Value35/1 -> Subtract2/1
  Unit Delay11/1 -> [VDID_DelayPKERNumerator_kphsqr]
  [VINP_CANMsgValidMCUBR1_flg] -> AND6/2
  Constant60/1 -> Divide/1
  [VDID_PKENumeratorOneSec_kphsqr] -> Subtract2/2
  [VTQD_VehActSpd_kph] -> Square/1, Delay/1
  [VDID_DelayPKELNumerator_kphsqr] -> Initial Value36/2
  [VDID_DelayPKELNumerator_kphsqr] -> Initial Value37/2
  [VDID_DelayPKERNumerator_kphsqr] -> Initial Value35/2
  Square/1 -> Minus/1
  Divide/1 -> Delay/2
  Square1/1 -> Minus/2
  [VINP_FlashPKERNumerator_kphsqr] -> Initial Value34/1
  Switch12/1 -> Unit Delay23/1, [VDID_PKELNumerator_kphsqr]
  Equal19/1 -> Switch11/2
  Subtract3/1 -> Switch12/1
  [VINP_FlashPKELNumerator_kphsqr] -> Initial Value36/1
  Max3/1 -> [VDID_PKENumeratorOneSec_kphsqr]
  Subtract2/1 -> Switch60/1
  [VINP_CANMsgValidESC1_flg] -> AND2/1
  Constant56/1 -> Switch10/1
  [VDID_DelayPKERNumerator_kphsqr] -> Initial Value34/2
  Constant46/1 -> Equal20/2
  Constant50/1 -> Switch16/3
  Switch11/1 -> [VDID_PKER_kphsqr]
  [VDID_CDEODTR_km] -> Equal19/1
  AND6/1 -> Scheduler/2(trigger)
  [VDID_CDEODTL_km] -> Divide2/2
  Initial Value37/1 -> Subtract3/1
  Scheduler1/1(trig_1sec) -> Switch12/2
  Equal20/1 -> Switch16/2
  Initial Value34/1 -> Switch60/3
  Constant21/1 -> Seconds_Counter/5
  Data Type Conversion12/1 -> [VDID_HVESSCHARGEACT_kW]
  [VTQD_VehActSpd_kph] -> 0xF819: Total Propulsion System Active Time/5(VTQD_VehActSpd_kph)
  [VINP_CANMsgValidESC1_flg] -> 0xF819: Total Propulsion System Active Time/6(VINP_CANMsgValidESC1_flg)
  [VINP_CANMsgValidMCUBR1_flg] -> 0xF819: Total Propulsion System Active Time/7(VINP_CANMsgValidMCUBR1_flg)
  [VDHP_LowIdleAccPedal_flg] -> 0xF819: Total Propulsion System Active Time/4(VDHP_LowIdleAccPedal_flg)
  [VINP_FlashPSAR_sec] -> 0xF819: Total Propulsion System Active Time/8(VINP_FlashPSAR_sec)
  [VINP_ClearDTCcmd_flg] -> 0xF819: Total Propulsion System Active Time/3(VINP_ClearDTCcmd_flg)
  [VINP_FlashPSAL_sec] -> 0xF819: Total Propulsion System Active Time/9(VINP_FlashPSAL_sec)
  [task_time_s] -> 0xF819: Total Propulsion System Active Time/2(task_time_s)
  [VPMM_SysPowerMode_enum] -> 0xF819: Total Propulsion System Active Time/1(VPMM_SysPowerMode_enum)
  [VINP_FlashIPSAR_sec] -> 0xF819: Total Propulsion System Active Time/10(VINP_FlashIPSAR_sec)
  [VINP_FlashIPSAL_sec] -> 0xF819: Total Propulsion System Active Time/11(VINP_FlashIPSAL_sec)
  [VINP_FlashCPSAR_sec] -> 0xF819: Total Propulsion System Active Time/12(VINP_FlashCPSAR_sec)
  [VINP_FlashCPSAL_sec] -> 0xF819: Total Propulsion System Active Time/13(VINP_FlashCPSAL_sec)
  0xF819: Total Propulsion System Active Time/5(VDID_IPSAL_sec) -> [VDID_IPSAL_sec]
  0xF819: Total Propulsion System Active Time/6(VDID_CPSAR_sec) -> [VDID_CPSAR_sec]
  0xF819: Total Propulsion System Active Time/4(VDID_IPSAR_sec) -> [VDID_IPSAR_sec]
  0xF819: Total Propulsion System Active Time/7(VDID_CPSAL_sec) -> [VDID_CPSAL_sec]
  0xF819: Total Propulsion System Active Time/3(VDID_PSAL_sec) -> [VDID_PSAL_sec]
  0xF819: Total Propulsion System Active Time/2(VDID_PSAR_sec) -> [VDID_PSAR_sec]
  0xF819: Total Propulsion System Active Time/1(VDID_NoteAResetCondition_flg) -> [VDID_NoteAResetCondition_flg]
  [VINP_FlashTNECPSAL_kWh] -> 0xF885 - 0xF88B/10(VINP_FlashTNECPSAL_kWh)
  [VINP_FlashTNECPSAR_kWh] -> 0xF885 - 0xF88B/9(VINP_FlashTNECPSAR_kWh)
  [VDID_HVBattPwrChrg_kW] -> 0xF885 - 0xF88B/11(VDID_HVBattPwrChrg_kW)
  [VDID_HVBattPwrDischrg_kW] -> 0xF885 - 0xF88B/8(VDID_HVBattPwrDischrg_kW)
  [VINP_ChrgPlugSta_enum] -> 0xF885 - 0xF88B/12(VINP_ChrgPlugSta_enum)
  [VINP_FlashTNBCPSAL_Ahr] -> 0xF885 - 0xF88B/7(VINP_FlashTNBCPSAL_Ahr)
  [VINP_FlashTEBPSAR_kWh] -> 0xF885 - 0xF88B/13(VINP_FlashTEBPSAR_kWh)
  [VDID_NoteAResetCondition_flg] -> 0xF885 - 0xF88B/6(VDID_NoteAResetCondition_flg)
  [VINP_CANMsgValidBMS1_flg] -> 0xF885 - 0xF88B/5(VINP_CANMsgValidBMS1_flg)
  [VINP_CANMsgValidBMS6_flg] -> 0xF885 - 0xF88B/14(VINP_CANMsgValidBMS6_flg)
  [VINP_FlashTNBCPSAR_Ahr] -> 0xF885 - 0xF88B/4(VINP_FlashTNBCPSAR_Ahr)
  [VINP_FlashTEBPSAL_kWh] -> 0xF885 - 0xF88B/15(VINP_FlashTEBPSAL_kWh)
  [VPMM_SysPowerMode_enum] -> 0xF885 - 0xF88B/3(VPMM_SysPowerMode_enum)
  [VINP_ExtChrgSta_enum] -> 0xF885 - 0xF88B/16(VINP_ExtChrgSta_enum)
  [task_time_s] -> 0xF885 - 0xF88B/2(task_time_s)
  [VINP_FlashTGEOVCR_kWh] -> 0xF885 - 0xF88B/17(VINP_FlashTGEOVCR_kWh)
  [VDID_HVBattCurr_A] -> 0xF885 - 0xF88B/1(VDID_HVBattCurr_A)
  [VINP_FlashTGEOVCL_kWh] -> 0xF885 - 0xF88B/18(VINP_FlashTGEOVCL_kWh)
  [VINP_FlashGECHGOVCDCR_kWh] -> 0xF885 - 0xF88B/19(VINP_FlashGECHGOVCDCR_kWh)
  [VINP_FlashGECHGOVCDCL_kWh] -> 0xF885 - 0xF88B/20(VINP_FlashGECHGOVCDCL_kWh)
  [VINP_FlashGECHGOVCACR_kWh] -> 0xF885 - 0xF88B/21(VINP_FlashGECHGOVCACR_kWh)
  [VINP_FlashGECHGOVCACL_kWh] -> 0xF885 - 0xF88B/22(VINP_FlashGECHGOVCACL_kWh)
  [VINP_FlashRESSV2XENNONPSAR_kWh] -> 0xF885 - 0xF88B/23(VINP_FlashRESSV2XENNONPSAR_kWh)
  [VINP_FlashRESSV2XENNONPSAL_kWh] -> 0xF885 - 0xF88B/24(VINP_FlashRESSV2XENNONPSAL_kWh)
  [VINP_CANMsgValidCCU2_flg] -> 0xF885 - 0xF88B/25(VINP_CANMsgValidCCU2_flg)
  0xF885 - 0xF88B/4(VDID_TNECPSAL_kWh) -> [VDID_TNECPSAL_kWh]
  0xF885 - 0xF88B/5(VDID_TEBPSAR_kWh) -> [VDID_TEBPSAR_kWh]
  0xF885 - 0xF88B/3(VDID_TNECPSAR_kWh) -> [VDID_TNECPSAR_kWh]
  0xF885 - 0xF88B/6(VDID_TEBPSAL_kWh) -> [VDID_TEBPSAL_kWh]
  0xF885 - 0xF88B/2(VDID_TNBCPSAL_Ahr) -> [VDID_TNBCPSAL_Ahr]
  0xF885 - 0xF88B/7(VDID_TGEOVCR_kWh) -> [VDID_TGEOVCR_kWh]
  0xF885 - 0xF88B/1(VDID_TNBCPSAR_Ahr) -> [VDID_TNBCPSAR_Ahr]
  0xF885 - 0xF88B/8(VDID_TGEOVCL_kWh) -> [VDID_TGEOVCL_kWh]
  0xF885 - 0xF88B/9(VDID_GECHGOVCDCR_kWh) -> [VDID_GECHGOVCDCR_kWh]
  0xF885 - 0xF88B/10(VDID_GECHGOVCDCL_kWh) -> [VDID_GECHGOVCDCL_kWh]
  0xF885 - 0xF88B/11(VDID_GECHGOVCACR_kWh) -> [VDID_GECHGOVCACR_kWh]
  0xF885 - 0xF88B/12(VDID_GECHGOVCACL_kWh) -> [VDID_GECHGOVCACL_kWh]
  0xF885 - 0xF88B/13(VDID_RESSV2XENNONPSAR_kWh) -> [VDID_RESSV2XENNONPSAR_kWh]
  0xF885 - 0xF88B/14(VDID_RESSV2XENNONPSAL_kWh) -> [VDID_RESSV2XENNONPSAL_kWh]
  [VINP_CellTempAvg_C] -> 0xF88E - 0xF890/7(VINP_CellTempAvg_C)
  [task_time_s] -> 0xF88E - 0xF890/6(task_time_s)
  [VINP_FlashTempPSAR_sec] -> 0xF88E - 0xF890/8(VINP_FlashTempPSAR_sec)
  [VINP_ChrgPlugSta_enum] -> 0xF88E - 0xF890/5(VINP_ChrgPlugSta_enum)
  [VDID_FlashAvgBattTempPSAR_C] -> 0xF88E - 0xF890/9(VDID_FlashAvgBattTempPSAR_C)
  [VINP_FlashTempPSAL_sec] -> 0xF88E - 0xF890/10(VINP_FlashTempPSAL_sec)
  [VDID_NoteAResetCondition_flg] -> 0xF88E - 0xF890/4(VDID_NoteAResetCondition_flg)
  [VINP_CANMsgValidBMS6_flg] -> 0xF88E - 0xF890/3(VINP_CANMsgValidBMS6_flg)
  [VDID_FlashAvgBattTempPSAL_C] -> 0xF88E - 0xF890/11(VDID_FlashAvgBattTempPSAL_C)
  [VINP_FlashOVCR_sec] -> 0xF88E - 0xF890/12(VINP_FlashOVCR_sec)
  [VINP_CANMsgValidBMS4_flg] -> 0xF88E - 0xF890/2(VINP_CANMsgValidBMS4_flg)
  [VPMM_SysPowerMode_enum] -> 0xF88E - 0xF890/1(VPMM_SysPowerMode_enum)
  [VDID_FlashAvgBattTempOVCR_C] -> 0xF88E - 0xF890/13(VDID_FlashAvgBattTempOVCR_C)
  [VINP_FlashOVCL_sec] -> 0xF88E - 0xF890/14(VINP_FlashOVCL_sec)
  [VDID_FlashAvgBattTempOVCL_C] -> 0xF88E - 0xF890/15(VDID_FlashAvgBattTempOVCL_C)
  [VINP_FlashOFFR_sec] -> 0xF88E - 0xF890/16(VINP_FlashOFFR_sec)
  [VDID_FlashAvgBattTempOFFR_C] -> 0xF88E - 0xF890/17(VDID_FlashAvgBattTempOFFR_C)
  [VINP_FlashOFFL_sec] -> 0xF88E - 0xF890/18(VINP_FlashOFFL_sec)
  [VDID_FlashAvgBattTempOFFL_C] -> 0xF88E - 0xF890/19(VDID_FlashAvgBattTempOFFL_C)
  0xF88E - 0xF890/2(VDID_AvgBattTempPSAL_C) -> [VDID_AvgBattTempPSAL_C]
  0xF88E - 0xF890/3(VDID_AvgBattTempOVCR_C) -> [VDID_AvgBattTempOVCR_C]
  0xF88E - 0xF890/1(VDID_AvgBattTempPSAR_C) -> [VDID_AvgBattTempPSAR_C]
  0xF88E - 0xF890/4(VDID_AvgBattTempOVCL_C) -> [VDID_AvgBattTempOVCL_C]
  0xF88E - 0xF890/5(VDID_AvgBattTempOFFR_C) -> [VDID_AvgBattTempOFFR_C]
  0xF88E - 0xF890/6(VDID_AvgBattTempOFFL_C) -> [VDID_AvgBattTempOFFL_C]
  VINP_FlashCPSAL_sec/1 -> [VINP_FlashCPSAL_sec]
  VINP_FlashCPSAR_sec/1 -> [VINP_FlashCPSAR_sec]
  VINP_FlashPSAL_sec/1 -> [VINP_FlashPSAL_sec]
  VINP_FlashIPSAR_sec/1 -> [VINP_FlashIPSAR_sec]
  VINP_FlashIPSAL_sec/1 -> [VINP_FlashIPSAL_sec]
  VINP_FlashPSAR_sec/1 -> [VINP_FlashPSAR_sec]
  VINP_FlashMILDIST_km/1 -> [VINP_FlashMILDIST_km]
  VINP_FlashWARMUPS_cnt/1 -> [VINP_FlashWARMUPS_cnt]
  VINP_FlashDelayCLRDIST_km/1 -> [VINP_FlashDelayCLRDIST_km]
  VINP_FlashMILTime_min/1 -> [VINP_FlashMILTime_min]
  VINP_FlashCLRTime_min/1 -> [VINP_FlashCLRTime_min]
  VINP_FlashNUMPSATRIPSFLTMEMCLR_cnt/1 -> [VINP_FlashNUMPSATRIPSFLTMEMCLR_cnt]
  VINP_FlashTNBCPSAL_Ahr/1 -> [VINP_FlashTNBCPSAL_Ahr]
  VINP_CANMsgValidBMS6_flg/1 -> [VINP_CANMsgValidBMS6_flg]
  VINP_FlashTEBPSAL_kWh/1 -> [VINP_FlashTEBPSAL_kWh]
  VINP_FlashTNECPSAR_kWh/1 -> [VINP_FlashTNECPSAR_kWh]
  VINP_FlashGECHGOVCACR_kWh/1 -> [VINP_FlashGECHGOVCACR_kWh]
  VINP_FlashTGEOVCL_kWh/1 -> [VINP_FlashTGEOVCL_kWh]
  VINP_FlashTGEOVCR_kWh/1 -> [VINP_FlashTGEOVCR_kWh]
  VINP_FlashGECHGOVCACL_kWh/1 -> [VINP_FlashGECHGOVCACL_kWh]
  VINP_FlashTEBPSAR_kWh/1 -> [VINP_FlashTEBPSAR_kWh]
  VINP_FlashGECHGOVCDCR_kWh/1 -> [VINP_FlashGECHGOVCDCR_kWh]
  VINP_FlashTNBCPSAR_Ahr/1 -> [VINP_FlashTNBCPSAR_Ahr]
  VINP_FlashRESSV2XENNONPSAL_kWh/1 -> [VINP_FlashRESSV2XENNONPSAL_kWh]
  VINP_FlashRESSV2XENNONPSAR_kWh/1 -> [VINP_FlashRESSV2XENNONPSAR_kWh]
  VINP_FlashTNECPSAL_kWh/1 -> [VINP_FlashTNECPSAL_kWh]
  VINP_FlashGECHGOVCDCL_kWh/1 -> [VINP_FlashGECHGOVCDCL_kWh]
  VINP_FlashIGNCNTR_cnt/1 -> [VINP_FlashIGNCNTR_cnt]
  VINP_FlashHVBNAH_Ah/1 -> [VINP_FlashHVBNAH_Ah]
  Unit Delay5/1 -> Initial Value4/2
  Initial Value4/1 -> Switch9/3
  [VINP_FlashODOMETER_km] -> Initial Value4/1
  VINP_FlashODOMETER_km/1 -> [VINP_FlashODOMETER_km]
  VINP_FlashPKERNumerator_kphsqr/1 -> [VINP_FlashPKERNumerator_kphsqr]
  VINP_FlashPKELNumerator_kphsqr/1 -> [VINP_FlashPKELNumerator_kphsqr]
  VINP_FlashResetCDEODTR_km/1 -> [VINP_FlashResetCDEODTR_km]
  VINP_FlashAvgBattTempOVCL_C/1 -> [VINP_FlashAvgBattTempOVCL_C]
  VINP_FlashOVCR_sec/1 -> [VINP_FlashOVCR_sec]
  VINP_FlashAvgBattTempPSAL_C/1 -> [VINP_FlashAvgBattTempPSAL_C]
  VINP_FlashTempPSAL_sec/1 -> [VINP_FlashTempPSAL_sec]
  VINP_FlashAvgBattTempOFFL_C/1 -> [VINP_FlashAvgBattTempOFFL_C]
  VINP_FlashAvgBattTempPSAR_C/1 -> [VINP_FlashAvgBattTempPSAR_C]
  VINP_FlashAvgBattTempOFFR_C/1 -> [VINP_FlashAvgBattTempOFFR_C]
  VINP_FlashTempPSAR_sec/1 -> [VINP_FlashTempPSAR_sec]
  VINP_FlashOVCL_sec/1 -> [VINP_FlashOVCL_sec]
  VINP_FlashOFFL_sec/1 -> [VINP_FlashOFFL_sec]
  VINP_FlashOFFR_sec/1 -> [VINP_FlashOFFR_sec]
  VINP_FlashAvgBattTempOVCR_C/1 -> [VINP_FlashAvgBattTempOVCR_C]
  Data Type Conversion7/1 -> [VDID_HEVBATT_V]
  [VDID_VSS_kph] -> VDID_VSS_kph/1  "VDID_VSS_kph"
  [VDID_RUNTM_s] -> VDID_RUNTM_s/1  "VDID_RUNTM_s"
  [VDID_MILDIST_km] -> VDID_MILDIST_km/1  "VDID_MILDIST_km"
  [VDID_WARMUPS_cnt] -> VDID_WARMUPS_cnt/1  "VDID_WARMUPS_cnt"
  [VDID_CLRDIST_km] -> VDID_CLRDIST_km/1  "VDID_CLRDIST_km"
  [VDID_APPD_pct] -> VDID_APPD_pct/1  "VDID_APPD_pct"
  [VDID_APPE_pct] -> VDID_APPE_pct/1  "VDID_APPE_pct"
  [VDID_MILTIME_min] -> VDID_MILTIME_min/1  "VDID_MILTIME_min"
  [VDID_CLRTIME_min] -> VDID_CLRTIME_min/1  "VDID_CLRTIME_min"
  [VDID_BATSOC_pct] -> VDID_BATSOC_pct/1  "VDID_BATSOC_pct"
  [VDID_HEVBATT_V] -> VDID_HEVBATT_V/1  "VDID_HEVBATT_V"
  [VDID_ODOMETER_km] -> VDID_ODOMETER_km/1  "VDID_ODOMETER_km"
  [VDID_BATSOH_pct] -> VDID_BATSOH_pct/1  "VDID_BATSOH_pct"
  [VDID_HVBCellVoltMin_V] -> VDID_HVBCellVoltMin_V/1  "VDID_HVBCellVoltMin_V"
  [VDID_HVBCellVoltMax_V] -> VDID_HVBCellVoltMax_V/1  "VDID_HVBCellVoltMax_V"
  [VDID_HVESSCHARGELIM_kW] -> VDID_HVESSCHARGELIM_kW/1  "VDID_HVESSCHARGELIM_kW"
  [VDID_HVESSCHARGEACT_kW] -> VDID_HVESSCHARGEACT_kW/1  "VDID_HVESSCHARGEACT_kW"
  [VDID_HVESSENER_Whps] -> VDID_HVESSENER_Whps/1  "VDID_HVESSENER_Whps"
  [VDID_NUMPSATRIPSFLTMEMCLR_cnt] -> VDID_NUMPSATRIPSFLTMEMCLR_cnt/1  "VDID_NUMPSATRIPSFLTMEMCLR_cnt"
  [VDID_HVBattCurr_Ahps] -> VDID_HVBattCurr_Ahps/1  "VDID_HVBattCurr_Ahps"
  [VDID_CPSAL_sec] -> VDID_CPSAL_sec/1  "VDID_CPSAL_sec"
  [VDID_CPSAR_sec] -> VDID_CPSAR_sec/1  "VDID_CPSAR_sec"
  [VDID_PSAR_sec] -> VDID_PSAR_sec/1  "VDID_PSAR_sec"
  [VDID_PSAL_sec] -> VDID_PSAL_sec/1  "VDID_PSAL_sec"
  [VDID_IPSAR_sec] -> VDID_IPSAR_sec/1  "VDID_IPSAR_sec"
  [VDID_IPSAL_sec] -> VDID_IPSAL_sec/1  "VDID_IPSAL_sec"
  Gain20/1 -> [VDID_HVBNAH_Ahr]
  Gain14/1 -> [VDID_HVBNE_kWh]
  [VDID_GECHGOVCDCL_kWh] -> VDID_GECHGOVCDCL_kWh/1  "VDID_GECHGOVCDCL_kWh"
  [VDID_TNBCPSAR_Ahr] -> VDID_TNBCPSAR_Ahr/1  "VDID_TNBCPSAR_Ahr"
  [VDID_GECHGOVCACR_kWh] -> VDID_GECHGOVCACR_kWh/1  "VDID_GECHGOVCACR_kWh"
  [VDID_RESSV2XENNONPSAR_kWh] -> VDID_RESSV2XENNONPSAR_kWh/1  "VDID_RESSV2XENNONPSAR_kWh"
  [VDID_TEBPSAR_kWh] -> VDID_TEBPSAR_kWh/1  "VDID_TEBPSAR_kWh"
  [VDID_TEBPSAL_kWh] -> VDID_TEBPSAL_kWh/1  "VDID_TEBPSAL_kWh"
  [VDID_TNECPSAL_kWh] -> VDID_TNECPSAL_kWh/1  "VDID_TNECPSAL_kWh"
  [VDID_TNECPSAR_kWh] -> VDID_TNECPSAR_kWh/1  "VDID_TNECPSAR_kWh"
  [VDID_GECHGOVCACL_kWh] -> VDID_GECHGOVCACL_kWh/1  "VDID_GECHGOVCACL_kWh"
  [VDID_TNBCPSAL_Ahr] -> VDID_TNBCPSAL_Ahr/1  "VDID_TNBCPSAL_Ahr"
  [VDID_TGEOVCR_kWh] -> VDID_TGEOVCR_kWh/1  "VDID_TGEOVCR_kWh"
  [VDID_GECHGOVCDCR_kWh] -> VDID_GECHGOVCDCR_kWh/1  "VDID_GECHGOVCDCR_kWh"
  [VDID_RESSV2XENNONPSAL_kWh] -> VDID_RESSV2XENNONPSAL_kWh/1  "VDID_RESSV2XENNONPSAL_kWh"
  [VDID_TGEOVCL_kWh] -> VDID_TGEOVCL_kWh/1  "VDID_TGEOVCL_kWh"
  [VDID_HVBNAH_Ahr] -> VDID_HVBNAH_Ahr/1  "VDID_HVBNAH_Ahr"
  [VDID_HVBNE_kWh] -> VDID_HVBNE_kWh/1  "VDID_HVBNE_kWh"
  [VDID_IGNCNTR_cnt] -> VDID_IGNCNTR_cnt/1  "VDID_IGNCNTR_cnt"
  [VDID_PKER_kphsqr] -> VDID_PKER_kphsqr/1  "VDID_PKER_kphsqr"
  [VDID_PKEL_kphsqr] -> VDID_PKEL_kphsqr/1  "VDID_PKEL_kphsqr"
  [VDID_ResetCDEODTR_km] -> VDID_ResetCDEODTR_km/1  "VDID_ResetCDEODTR_km"
  [VDID_CDEODTR_km] -> VDID_CDEODTR_km/1  "VDID_CDEODTR_km"
  [VDID_CDEODTL_km] -> VDID_CDEODTL_km/1  "VDID_CDEODTL_km"
  [VDID_AvgBattTempOFFR_C] -> VDID_AvgBattTempOFFR_C/1  "VDID_AvgBattTempOFFR_C"
  [VDID_AvgBattTempOFFL_C] -> VDID_AvgBattTempOFFL_C/1  "VDID_AvgBattTempOFFL_C"
  [VDID_AvgBattTempPSAL_C] -> VDID_AvgBattTempPSAL_C/1  "VDID_AvgBattTempPSAL_C"
  [VDID_AvgBattTempPSAR_C] -> VDID_AvgBattTempPSAR_C/1  "VDID_AvgBattTempPSAR_C"
  [VDID_AvgBattTempOVCR_C] -> VDID_AvgBattTempOVCR_C/1  "VDID_AvgBattTempOVCR_C"
  [VDID_AvgBattTempOVCL_C] -> VDID_AvgBattTempOVCL_C/1  "VDID_AvgBattTempOVCL_C"
  VINP_FlashHVBNE_kWh/1 -> [VINP_FlashHVBNE_kWh]
  VINP_CANMsgValidBMS1_flg/1 -> [VINP_CANMsgValidBMS1_flg]
  VINP_CANMsgValidCCU2_flg/1 -> [VINP_CANMsgValidCCU2_flg]
  VINP_CANMsgValidBMS4_flg/1 -> [VINP_CANMsgValidBMS4_flg]
  VINP_CellTempAvg_C/1 -> [VINP_CellTempAvg_C]
  Data Type Conversion13/1 -> [VDID_CDEODTL_km]
  [VINP_CANMsgValidMETER1_flg] -> Logical Operator1/2
  Subtract1/1 -> Add2/2
  Max1/1 -> Unit Delay4/1, [VDID_CLRDIST_km]
  Constant17/1 -> Data Type Conversion3/1
  Data Type Conversion3/1 -> Max1/2
  Constant4/1 -> Data Type Conversion2/1
  Data Type Conversion2/1 -> Max/2
  Saturation/1 -> [VDID_APPD_pct]
  [VINP_ClearDTCcmd_flg] -> Logical Operator7/2
  NOT2/1 -> Logical Operator7/1
  Logical Operator7/1 -> Minutes_Counter/2
  Unit Delay7/1 -> [VDID_DelayNUMPSATRIPSFLTMEMCLR_cnt]
  Switch6/1 -> Switch5/3
  Switch5/1 -> Unit Delay7/1, [VDID_NUMPSATRIPSFLTMEMCLR_cnt]
  Initial Value5/1 -> Switch6/3
  [VDID_DelayNUMPSATRIPSFLTMEMCLR_cnt] -> Initial Value5/2
  [VINP_FlashNUMPSATRIPSFLTMEMCLR_cnt] -> Initial Value5/1
  [VINP_FlashNUMPSATRIPSFLTMEMCLR_cnt] -> Initial Value6/1
  [VDID_DelayNUMPSATRIPSFLTMEMCLR_cnt] -> Initial Value6/2
  Initial Value6/1 -> Add3/1
  VINP_OBCV2LSta_enum/1 -> [VINP_OBCV2LSta_enum]
  [VINP_OBCV2LSta_enum] -> 0xF885 - 0xF88B/26(VINP_OBCV2LSta_enum)
  Logical Operator4/1 -> NOT4/1, Timer6/1
  Equal9/1 -> Logical Operator4/1
  NOT3/1 -> Logical Operator4/2
  [VPMM_SysPowerMode_enum] -> Equal13/1
  Constant26/1 -> Equal13/2
  Equal13/1 -> Detect Increase1/1
  Detect Increase1/1 -> Initializable_U32counter/1
  Initializable_U32counter/1 -> [VDID_QTYPSATRIPSR_cnt]
  Constant33/1 -> Initializable_U32counter/3
  [VDID_NoteAResetCondition_flg] -> Initializable_U32counter/2
  [VINP_FlashQTYPSATRIPSR_cnt] -> Initializable_U32counter/4
  [VINP_FlashQTYPSATRIPSL_cnt] -> Initializable_U32counter1/4
  Constant35/1 -> Initializable_U32counter1/3
  Initializable_U32counter1/1 -> [VDID_QTYPSATRIPSL_cnt]
  Detect Increase3/1 -> Initializable_U32counter1/1
  Equal15/1 -> Detect Increase3/1
  Constant34/1 -> Equal15/2
  [VPMM_SysPowerMode_enum] -> Equal15/1
  Ground/1 -> Initializable_U32counter1/2
  VINP_FlashQTYPSATRIPSR_cnt/1 -> [VINP_FlashQTYPSATRIPSR_cnt]
  VINP_FlashQTYPSATRIPSL_cnt/1 -> [VINP_FlashQTYPSATRIPSL_cnt]
  [VDID_QTYPSATRIPSR_cnt] -> VDID_QTYPSATRIPSR_cnt/1  "VDID_QTYPSATRIPSR_cnt"
  [VDID_QTYPSATRIPSL_cnt] -> VDID_QTYPSATRIPSL_cnt/1  "VDID_QTYPSATRIPSL_cnt"
  [VDID_AVGBATTEMPL_C] -> VDID_AVGBATTEMPL_C/1  "VDID_AVGBATTEMPL_C"
  [VDID_MINBATTEMPL_C] -> VDID_MINBATTEMPL_C/1  "VDID_MINBATTEMPL_C"
  [VDID_RESSTIMESOCPSARNGR_s] -> VDID_RESSTIMESOCPSARNGR_s/1  "VDID_RESSTIMESOCPSARNGR_s"
  [VDID_RESSTIMESOCOFFRNGL_s] -> VDID_RESSTIMESOCOFFRNGL_s/1  "VDID_RESSTIMESOCOFFRNGL_s"
  [VDID_RESSTIMESOCCHGRNGR_s] -> VDID_RESSTIMESOCCHGRNGR_s/1  "VDID_RESSTIMESOCCHGRNGR_s"
  [VDID_ETMATOER_kWh] -> VDID_ETMATOER_kWh/1  "VDID_ETMATOER_kWh"
  [VDID_RESSTIMESOCPSARNGL_s] -> VDID_RESSTIMESOCPSARNGL_s/1  "VDID_RESSTIMESOCPSARNGL_s"
  [VDID_ETMBTOER_kWh] -> VDID_ETMBTOER_kWh/1  "VDID_ETMBTOER_kWh"
  [VDID_MAXBATTEMPL_C] -> VDID_MAXBATTEMPL_C/1  "VDID_MAXBATTEMPL_C"
  [VDID_RESSCNTDODRNGR_cnt] -> VDID_RESSCNTDODRNGR_cnt/1  "VDID_RESSCNTDODRNGR_cnt"
  [VDID_RESSTIMESOCCHGRNGL_s] -> VDID_RESSTIMESOCCHGRNGL_s/1  "VDID_RESSTIMESOCCHGRNGL_s"
  [VDID_ETMATOEL_kWh] -> VDID_ETMATOEL_kWh/1  "VDID_ETMATOEL_kWh"
  [VDID_RESSTIMESOCOFFRNGR_s] -> VDID_RESSTIMESOCOFFRNGR_s/1  "VDID_RESSTIMESOCOFFRNGR_s"
  [VDID_RESSCNTDODRNGL_cnt] -> VDID_RESSCNTDODRNGL_cnt/1  "VDID_RESSCNTDODRNGL_cnt"
  [VDID_ETMBTOEL_kWh] -> VDID_ETMBTOEL_kWh/1  "VDID_ETMBTOEL_kWh"
  0xF898-0xF8/1(VDID_RESSCNTDODRNGR_cnt) -> [VDID_RESSCNTDODRNGR_cnt]
  0xF898-0xF8/15(VDID_AVGBATTEMPL_C) -> [VDID_AVGBATTEMPL_C]
  0xF898-0xF8/14(VDID_MINBATTEMPL_C) -> [VDID_MINBATTEMPL_C]
  0xF898-0xF8/13(VDID_MAXBATTEMPL_C) -> [VDID_MAXBATTEMPL_C]
  0xF898-0xF8/12(VDID_RESSTIMESOCOFFRNGL_s) -> [VDID_RESSTIMESOCOFFRNGL_s]
  0xF898-0xF8/11(VDID_RESSTIMESOCOFFRNGR_s) -> [VDID_RESSTIMESOCOFFRNGR_s]
  0xF898-0xF8/10(VDID_RESSTIMESOCCHGRNGL_s) -> [VDID_RESSTIMESOCCHGRNGL_s]
  0xF898-0xF8/9(VDID_RESSTIMESOCCHGRNGR_s) -> [VDID_RESSTIMESOCCHGRNGR_s]
  0xF898-0xF8/8(VDID_RESSTIMESOCPSARNGL_s) -> [VDID_RESSTIMESOCPSARNGL_s]
  0xF898-0xF8/7(VDID_RESSTIMESOCPSARNGR_s) -> [VDID_RESSTIMESOCPSARNGR_s]
  0xF898-0xF8/6(VDID_ETMBTOEL_kWh) -> [VDID_ETMBTOEL_kWh]
  0xF898-0xF8/5(VDID_ETMBTOER_kWh) -> [VDID_ETMBTOER_kWh]
  0xF898-0xF8/4(VDID_ETMATOEL_kWh) -> [VDID_ETMATOEL_kWh]
  0xF898-0xF8/3(VDID_ETMATOER_kWh) -> [VDID_ETMATOER_kWh]
  0xF898-0xF8/2(VDID_RESSCNTDODRNGL_cnt) -> [VDID_RESSCNTDODRNGL_cnt]
  [VDID_HVBattPwr_kW] -> 0xF898-0xF8/1(VDID_HVBattPwr_kW)
  [VDID_NoteAResetCondition_flg] -> 0xF898-0xF8/4(VDID_NoteAResetCondition_flg)
  [VINP_FlashRESSCNTDODRNGR_cnt] -> 0xF898-0xF8/5(VINP_FlashRESSCNTDODRNGR_cnt)
  [task_time_s] -> 0xF898-0xF8/2(task_time_s)
  [VINP_CANMsgValidBMS1_flg] -> 0xF898-0xF8/3(VINP_CANMsgValidBMS1_flg)
  [VINP_FlashRESSCNTDODRNGL_cnt] -> 0xF898-0xF8/6(VINP_FlashRESSCNTDODRNGL_cnt)
  [VINP_FlashETMATOEL_kWh] -> 0xF898-0xF8/10(VINP_FlashETMATOEL_kWh)
  [VINP_RrMCUDCBusCurr_A] -> 0xF898-0xF8/7(VINP_RrMCUDCBusCurr_A)
  [VINP_RrMCUDCBusVolt_V] -> 0xF898-0xF8/8(VINP_RrMCUDCBusVolt_V)
  [VINP_FlashETMATOER_kWh] -> 0xF898-0xF8/9(VINP_FlashETMATOER_kWh)
  [VINP_CANMsgValidMCUBR1_flg] -> 0xF898-0xF8/11(VINP_CANMsgValidMCUBR1_flg)
  [VINP_FrMCUDCBusCurr_A] -> 0xF898-0xF8/12(VINP_FrMCUDCBusCurr_A)
  [VINP_FrMCUDCBusVolt_V] -> 0xF898-0xF8/13(VINP_FrMCUDCBusVolt_V)
  [VINP_FlashETMBTOER_kWh] -> 0xF898-0xF8/14(VINP_FlashETMBTOER_kWh)
  [VINP_FlashETMBTOEL_kWh] -> 0xF898-0xF8/15(VINP_FlashETMBTOEL_kWh)
  [VINP_FlashRESSTIMESOCPSARNGR_s] -> 0xF898-0xF8/21(VINP_FlashRESSTIMESOCPSARNGR_s)
  [VINP_CANMsgValidMCUBF1_flg] -> 0xF898-0xF8/16(VINP_CANMsgValidMCUBF1_flg)
  [VINP_HVBattSOC_pct] -> 0xF898-0xF8/20(VINP_HVBattSOC_pct)
  [VPMM_SysPowerMode_enum] -> 0xF898-0xF8/17(VPMM_SysPowerMode_enum)
  [VINP_FlashRESSTIMESOCPSARNGL_s] -> 0xF898-0xF8/22(VINP_FlashRESSTIMESOCPSARNGL_s)
  [VINP_ChrgPlugSta_enum] -> 0xF898-0xF8/18(VINP_ChrgPlugSta_enum)
  [VINP_ExtChrgSta_enum] -> 0xF898-0xF8/23(VINP_ExtChrgSta_enum)
  [VINP_CANMsgValidBMS6_flg] -> 0xF898-0xF8/19(VINP_CANMsgValidBMS6_flg)
  [VINP_FlashRESSTIMESOCCHGRNGR_s] -> 0xF898-0xF8/24(VINP_FlashRESSTIMESOCCHGRNGR_s)
  [VINP_FlashRESSTIMESOCCHGRNGL_s] -> 0xF898-0xF8/25(VINP_FlashRESSTIMESOCCHGRNGL_s)
  [VDID_FlashMAXBATTEMPL_C] -> 0xF898-0xF8/28(VDID_FlashMAXBATTEMPL_C)
  [VINP_FlashRESSTIMESOCOFFRNGL_s] -> 0xF898-0xF8/27(VINP_FlashRESSTIMESOCOFFRNGL_s)
  [VINP_HVBMTempMax_C] -> 0xF898-0xF8/29(VINP_HVBMTempMax_C)
  [VINP_FlashRESSTIMESOCOFFRNGR_s] -> 0xF898-0xF8/26(VINP_FlashRESSTIMESOCOFFRNGR_s)
  [VINP_CANMsgValidMETER1_flg] -> 0xF898-0xF8/30(VINP_CANMsgValidMETER1_flg)
  [VINP_HVBMTempMin_C] -> 0xF898-0xF8/32(VINP_HVBMTempMin_C)
  [VDID_FlashMINBATTEMPL_C] -> 0xF898-0xF8/31(VDID_FlashMINBATTEMPL_C)
  [VINP_FlashAVGBATTEMPL_sec] -> 0xF898-0xF8/34(VINP_FlashAVGBATTEMPL_sec)
  [VINP_CANMsgValidBMS4_flg] -> 0xF898-0xF8/33(VINP_CANMsgValidBMS4_flg)
  [VDID_FlashAVGBATTEMPL_C] -> 0xF898-0xF8/35(VDID_FlashAVGBATTEMPL_C)
  [VINP_CellTempAvg_C] -> 0xF898-0xF8/36(VINP_CellTempAvg_C)
  VINP_FlashRESSCNTDODRNGR_cnt/1 -> [VINP_FlashRESSCNTDODRNGR_cnt]
  VINP_FlashRESSCNTDODRNGL_cnt/1 -> [VINP_FlashRESSCNTDODRNGL_cnt]
  VINP_RrMCUDCBusCurr_A/1 -> [VINP_RrMCUDCBusCurr_A]
  VINP_RrMCUDCBusVolt_V/1 -> [VINP_RrMCUDCBusVolt_V]
  VINP_FlashETMATOER_kWh/1 -> [VINP_FlashETMATOER_kWh]
  VINP_FlashETMATOEL_kWh/1 -> [VINP_FlashETMATOEL_kWh]
  VINP_FlashAVGBATTEMPL_C/1 -> [VINP_FlashAVGBATTEMPL_C]
  VINP_FlashAVGBATTEMPL_sec/1 -> [VINP_FlashAVGBATTEMPL_sec]
  VINP_FlashMINBATTEMPL_C/1 -> [VINP_FlashMINBATTEMPL_C]
  VINP_HVBMTempMax_C/1 -> [VINP_HVBMTempMax_C]
  VINP_HVBMTempMin_C/1 -> [VINP_HVBMTempMin_C]
  VINP_FlashMAXBATTEMPL_C/1 -> [VINP_FlashMAXBATTEMPL_C]
  VINP_FlashRESSTIMESOCOFFRNGL_s/1 -> [VINP_FlashRESSTIMESOCOFFRNGL_s]
  VINP_FlashRESSTIMESOCOFFRNGR_s/1 -> [VINP_FlashRESSTIMESOCOFFRNGR_s]
  VINP_FlashRESSTIMESOCCHGRNGL_s/1 -> [VINP_FlashRESSTIMESOCCHGRNGL_s]
  VINP_FlashRESSTIMESOCCHGRNGR_s/1 -> [VINP_FlashRESSTIMESOCCHGRNGR_s]
  VINP_FlashRESSTIMESOCPSARNGL_s/1 -> [VINP_FlashRESSTIMESOCPSARNGL_s]
  VINP_FlashRESSTIMESOCPSARNGR_s/1 -> [VINP_FlashRESSTIMESOCPSARNGR_s]
  VINP_CANMsgValidMCUBF1_flg/1 -> [VINP_CANMsgValidMCUBF1_flg]
  VINP_FlashETMBTOEL_kWh/1 -> [VINP_FlashETMBTOEL_kWh]
  VINP_FlashETMBTOER_kWh/1 -> [VINP_FlashETMBTOER_kWh]
  VINP_FrMCUDCBusVolt_V/1 -> [VINP_FrMCUDCBusVolt_V]
  VINP_FrMCUDCBusCurr_A/1 -> [VINP_FrMCUDCBusCurr_A]
  Constant36/1 -> Data Type Conversion4/1
  [VDID_PROTOCOLID_enum] -> VDID_PRO TOCOLID_enum/1  "VDID_PROTOCOLID_enum"
  Data Type Conversion4/1 -> [VDID_PROTOCOLID_enum]
  [VDID_HVBattPwrDischrg_kW] -> 0xF898-0xF8/37(VDID_HVBattPwrDischrg_kW)
  VINP_CANMsgValidBMS3_flg/1 -> [VINP_CANMsgValidBMS3_flg]
  VINP_MCUBFRealPwrKwSta_kW/1 -> [VINP_MCUBFRealPwrKwSta_kW]
  VINP_MCUBRRealPwrKwSta_kW/1 -> [VINP_MCUBRRealPwrKwSta_kW]
  [VINP_MCUBRRealPwrKwSta_kW] -> 0xF898-0xF8/38(VINP_MCUBRRealPwrKwSta_kW)
  [VINP_MCUBFRealPwrKwSta_kW] -> 0xF898-0xF8/39(VINP_MCUBFRealPwrKwSta_kW)
  [VINP_CANMsgValidBMS3_flg] -> 0xF898-0xF8/40(VINP_CANMsgValidBMS3_flg)
  0xF898-0xF8/16(VDID_RESSTTEMPRNGAXIS_enum) -> [VDID_RESSTTEMPRNGAXIS_enum]
  0xF898-0xF8/17(VDID_RESSTIMESOCRNGAXIS_enum) -> [VDID_RESSTIMESOCRNGAXIS_enum]
  0xF898-0xF8/18(VDID_RESSCNTSDODRNGAXIS_enum) -> [VDID_RESSCNTSDODRNGAXIS_enum]
  [VDID_RESSTIMESOCRNGAXIS_enum] -> VDID_RESSTIMESOCRNGAXIS_enum/1  "VDID_RESSTIMESOCRNGAXIS_enum"
  [VDID_RESSCNTSDODRNGAXIS_enum] -> VDID_RESSCNTSDODRNGAXIS_enum/1  "VDID_RESSCNTSDODRNGAXIS_enum"
  [VDID_RESSTTEMPRNGAXIS_enum] -> VDID_RESSTTEMPRNGAXIS_enum/1  "VDID_RESSTTEMPRNGAXIS_enum"
  String to ASCII2/1 -> Mux/3
  String Constant2/1 -> String to ASCII2/1
  String Constant/1 -> String to ASCII/1
  String to ASCII1/1 -> Mux/2
  String Constant1/1 -> String to ASCII1/1
  String to ASCII/1 -> Mux/1
  VINP_VehicleType_enum/1 -> [VINP_VehicleType_enum]
  VINP_CarModel1_cnt/1 -> [VINP_CarModel1_cnt]
  VINP_CarModel2_cnt/1 -> [VINP_CarModel2_cnt]
  VINP_ECU2_cnt/1 -> [VINP_ECU2_cnt]
  VINP_ECU1_cnt/1 -> [VINP_ECU1_cnt]
  VINP_CarModel3_cnt/1 -> [VINP_CarModel3_cnt]
  VINP_Major1_cnt/1 -> [VINP_Major1_cnt]
  VINP_Major2_cnt/1 -> [VINP_Major2_cnt]
  VINP_Minor1_cnt/1 -> [VINP_Minor1_cnt]
  VINP_ECUGen2_cnt/1 -> [VINP_ECUGen2_cnt]
  VINP_ECUGen1_cnt/1 -> [VINP_ECUGen1_cnt]
  VINP_Variation_cnt/1 -> [VINP_Variation_cnt]
  VINP_Patch2_cnt/1 -> [VINP_Patch2_cnt]
  VINP_Country1_cnt/1 -> [VINP_Country1_cnt]
  VINP_Country2_cnt/1 -> [VINP_Country2_cnt]
  VINP_Patch1_cnt/1 -> [VINP_Patch1_cnt]
  VINP_Minor2_cnt/1 -> [VINP_Minor2_cnt]
  [VINP_CarModel3_cnt] -> Mux1/3
  [VINP_CarModel2_cnt] -> Mux1/2
  [VINP_CarModel1_cnt] -> Mux1/1
  [VDID_CALID_cnt] -> VDID_CALID_cnt/1  "VDID_CALID_cnt"
  [VDID_ECUNAME_cnt] -> VDID_ECUNAME_cnt/1  "VDID_ECUNAME_cnt"
  [VDID_PKERNumerator_kphsqr] -> VDID_PKERNumerator_kphsqr/1  "VDID_PKERNumerator_kphsqr"
  [VDID_PKELNumerator_kphsqr] -> VDID_PKELNumerator_kphsqr/1  "VDID_PKELNumerator_kphsqr"
  [VDID_BattTempPSAL_sec] -> VDID_BattTempPSAL_sec/1  "VDID_BattTempPSAL_sec"
  [VDID_BattTempPSAR_sec] -> VDID_BattTempPSAR_sec/1  "VDID_BattTempPSAR_sec"
  [VDID_OVCL_sec] -> VDID_OVCL_sec/1  "VDID_OVCL_sec"
  [VDID_OVCR_sec] -> VDID_OVCR_sec/1  "VDID_OVCR_sec"
  [VDID_OFFR_sec] -> VDID_OFFR_sec/1  "VDID_OFFR_sec"
  [VDID_OFFL_sec] -> VDID_OFFL_sec/1  "VDID_OFFL_sec"
  [VDID_AVGBATTEMPL_sec] -> VDID_AVGBATTEMPL_sec/1  "VDID_AVGBATTEMPL_sec"
  0xF898-0xF8/19(VDID_AVGBATTEMPL_sec) -> [VDID_AVGBATTEMPL_sec]
  0xF88E - 0xF890/7(VDID_BattTempPSAR_sec) -> [VDID_BattTempPSAR_sec]
  0xF88E - 0xF890/8(VDID_BattTempPSAL_sec) -> [VDID_BattTempPSAL_sec]
  0xF88E - 0xF890/9(VDID_OVCR_sec) -> [VDID_OVCR_sec]
  0xF88E - 0xF890/10(VDID_OVCL_sec) -> [VDID_OVCL_sec]
  0xF88E - 0xF890/11(VDID_OFFR_sec) -> [VDID_OFFR_sec]
  0xF88E - 0xF890/12(VDID_OFFL_sec) -> [VDID_OFFL_sec]
  Mux1/1 -> Data Type Conversion5/1
  Data Type Conversion5/1 -> [VDID_CALID_cnt]
  Mux/1 -> Data Type Conversion11/1
  [VINP_Major1_cnt] -> Mux1/4
  [VINP_Major2_cnt] -> Mux1/5
  [VINP_Minor1_cnt] -> Mux1/6
  [VINP_Minor2_cnt] -> Mux1/7
  [VINP_Patch1_cnt] -> Mux1/8
  [VINP_Patch2_cnt] -> Mux1/9
  [VINP_Country1_cnt] -> Mux1/10
  [VINP_Country2_cnt] -> Mux1/11
  [VINP_Variation_cnt] -> Mux1/12
  [VINP_ECUGen1_cnt] -> Mux1/13
  [VINP_ECUGen2_cnt] -> Mux1/14
  VPMM_DrivetrainSelect_enum/1 -> [VPMM_DrivetrainSelect_enum]
  [VDID_DrivingMode_cnt] -> Mux1/15
  [VPMM_DrivetrainSelect_enum] -> 1-D Lookup Table/1
  [VPMM_DrivetrainSelect_enum] -> Equal16/1
  Constant39/1 -> Equal16/2
  Constant40/1 -> Equal17/2
  [VPMM_DrivetrainSelect_enum] -> Equal17/1
  [VPMM_DrivetrainSelect_enum] -> Equal21/1
  Constant41/1 -> Equal21/2
  Equal16/1 -> OR/1
  Equal17/1 -> OR/2
  Equal21/1 -> OR/3
  OR/1 -> Switch7/2
  1-D Lookup Table/1 -> Switch7/1
  Switch7/1 -> [VDID_DrivingMode_cnt]
  String to ASCII3/1 -> Switch7/3
  String Constant3/1 -> String to ASCII3/1
  [VDID_ModelYear_cnt] -> Mux1/16
  String Constant4/1 -> String to ASCII4/1
  String to ASCII4/1 -> [VDID_ModelYear_cnt]
  VINP_VinCode_cnt/1 -> [VINP_VinCode_cnt]
  [VINP_VinCode_cnt] -> Data Type Conversion14/1
  Data Type Conversion14/1 -> [VDID_VinCode_cnt]
  [VDID_VinCode_cnt] -> VDID_VinCode_cnt/1  "VDID_VinCode_cnt"
  [VDID_DelayCLRDIST_km] -> Add2/1
  Initial Value/1 -> Switch4/3
  Add2/1 -> Initial Value/2
  [VINP_FlashDelayCLRDIST_km] -> Initial Value/1
  Constant45/1 -> Shift Arithmetic313/1
  Shift Arithmetic313/1 -> Bitwise OR123/4
  Constant44/1 -> Shift Arithmetic312/1
  Constant42/1 -> Bitwise OR123/1
  Shift Arithmetic312/1 -> Bitwise OR123/3
  Constant43/1 -> Shift Arithmetic311/1
  Shift Arithmetic311/1 -> Bitwise OR123/2
  Shift Arithmetic1/1 -> Bitwise OR123/5
  Shift Arithmetic2/1 -> Bitwise OR123/6
  Shift Arithmetic3/1 -> Bitwise OR123/7
  Shift Arithmetic4/1 -> Bitwise OR123/8
  Constant47/1 -> Shift Arithmetic1/1
  Constant48/1 -> Shift Arithmetic2/1
  Constant51/1 -> Shift Arithmetic3/1
  Constant52/1 -> Shift Arithmetic4/1
  Constant63/1 -> Shift Arithmetic11/1
  Constant62/1 -> Shift Arithmetic7/1
  Constant61/1 -> Shift Arithmetic6/1
  Constant58/1 -> Shift Arithmetic5/1
  Shift Arithmetic8/1 -> Bitwise OR1/2
  Constant53/1 -> Bitwise OR1/1
  Constant57/1 -> Shift Arithmetic10/1
  Shift Arithmetic11/1 -> Bitwise OR1/7
  Shift Arithmetic7/1 -> Bitwise OR1/6
  Shift Arithmetic6/1 -> Bitwise OR1/5
  Shift Arithmetic5/1 -> Bitwise OR1/4
  Shift Arithmetic10/1 -> Bitwise OR1/3
  Data Type Conversion15/1 -> [VDID_HVBATT_A]
  [VDID_HVBattCurr_A] -> Data Type Conversion15/1
  Bitwise OR1/1 -> Data Type Conversion17/1
  Bitwise OR123/1 -> Data Type Conversion16/1
  Constant54/1 -> Shift Arithmetic8/1
  [VDID_STASUP_enum] -> VDID_STASUP_enum/1  "VDID_STASUP_enum"
  [VDID_HEVMODE_enum] -> VDID_HEVMODE_enum/1  "VDID_HEVMODE_enum"
  [VDID_HVBATT_A] -> VDID_HVBATT_A/1  "VDID_HVBATT_A"
  Data Type Conversion16/1 -> [VDID_STASUP_enum]
  Data Type Conversion17/1 -> [VDID_HEVMODE_enum]
  Data Type Conversion11/1 -> Reshape/1
  Reshape/1 -> [VDID_ECUNAME_cnt]
  Add/1 -> Initial Value2/2
  Initial Value2/1 -> Switch/1
  NOT4/1 -> Timer6/2
  Subsystem/1(VDID_DIDModelVersion_raw) -> [VDID_DIDModelVersion_raw]
  Cast To Boolean/1 -> Subsystem/Enable
  Subsystem/2(VDID_DIDModelVersionChksum_raw) -> [VDID_DIDModelVersionChksum_raw]
  Constant64/1 -> Delay1/1
  Logical Operator8/1 -> Cast To Boolean/1
  Delay1/1 -> Logical Operator8/1
  VINP_FlashModelVersion_raw/1 -> [VINP_FlashModelVersion_raw]
  VINP_FlashModelVersionChksum_raw/1 -> [VINP_FlashModelVersionChksum_raw]
  [VINP_FlashModelVersion_raw] -> Checksum/1(ModelVersion)
  [VINP_FlashModelVersionChksum_raw] -> Equal22/2
  Constant55/1 -> Equal23/2
  [VDID_DIDModelVersion_raw] -> Equal23/1
  Equal23/1 -> Logical Operator9/1
  Checksum/1(ModelVersionChksum) -> Equal22/1
  Equal22/1 -> [VDID_ModelVersionChksumValid_flg]
  [VDID_ModelVersionChksumValid_flg] -> Logical Operator9/2
  Logical Operator9/1 -> [VDID_FlashValid_flg]
  [VDID_DIDModelVersionChksum_raw] -> VDID_DIDModelVersionChksum_raw/1  "VDID_DIDModelVersionChksum_raw"
  [VDID_DIDModelVersion_raw] -> VDID_DIDModelVersion_raw/1  "VDID_DIDModelVersion_raw"
  [VINP_FlashHVBNAH_Ah] -> Switch14/1
  [VDID_FlashValid_flg] -> Switch14/2
  Constant65/1 -> Switch14/3
  Switch14/1 -> [VDID_FlashHVBNAH_Ah]
  Switch15/1 -> [VDID_FlashHVBNE_kWh]
  Constant68/1 -> Switch15/3
  [VDID_FlashValid_flg] -> Switch15/2
  [VINP_FlashHVBNE_kWh] -> Switch15/1
  [VDID_FlashValid_flg] -> Switch17/2
  Constant69/1 -> Switch17/3
  Constant72/1 -> Switch20/3
  [VDID_FlashValid_flg] -> Switch20/2
  [VDID_FlashValid_flg] -> Switch19/2
  Constant71/1 -> Switch19/3
  Constant70/1 -> Switch18/3
  [VDID_FlashValid_flg] -> Switch18/2
  Constant73/1 -> Switch23/3
  [VDID_FlashValid_flg] -> Switch23/2
  [VDID_FlashValid_flg] -> Switch24/2
  Constant74/1 -> Switch24/3
  [VINP_FlashAvgBattTempPSAR_C] -> Switch17/1
  [VINP_FlashAvgBattTempPSAL_C] -> Switch18/1
  [VINP_FlashAvgBattTempOVCR_C] -> Switch19/1
  [VINP_FlashAvgBattTempOVCL_C] -> Switch20/1
  [VINP_FlashAvgBattTempOFFR_C] -> Switch23/1
  [VINP_FlashAvgBattTempOFFL_C] -> Switch24/1
  Switch17/1 -> [VDID_FlashAvgBattTempPSAR_C]
  Switch18/1 -> [VDID_FlashAvgBattTempPSAL_C]
  Switch19/1 -> [VDID_FlashAvgBattTempOVCR_C]
  Switch20/1 -> [VDID_FlashAvgBattTempOVCL_C]
  Switch23/1 -> [VDID_FlashAvgBattTempOFFR_C]
  Switch24/1 -> [VDID_FlashAvgBattTempOFFL_C]
  Constant75/1 -> Switch25/3
  [VDID_FlashValid_flg] -> Switch25/2
  [VINP_FlashMAXBATTEMPL_C] -> Switch25/1
  [VDID_FlashValid_flg] -> Switch26/2
  Constant76/1 -> Switch26/3
  [VINP_FlashMINBATTEMPL_C] -> Switch26/1
  Constant77/1 -> Switch27/3
  [VDID_FlashValid_flg] -> Switch27/2
  [VINP_FlashAVGBATTEMPL_C] -> Switch27/1
  Switch25/1 -> [VDID_FlashMAXBATTEMPL_C]
  Switch26/1 -> [VDID_FlashMINBATTEMPL_C]
  Switch27/1 -> [VDID_FlashAVGBATTEMPL_C]
  Latch2/1 -> Unit Delay8/1
  Unit Delay9/1 -> Initial Value9/2
  From379/1 -> Detect Increase4/1
  From369/1 -> Minus3/2
  Minus4/1 -> Switch31/1
  Unit Delay8/1 -> Switch28/2
  Unit Delay3/1 -> Switch28/1
  Detect Increase4/1 -> Latch2/1
  From378/1 -> Minus4/2
  Switch28/1 -> Unit Delay3/1, Goto251/1
  From371/1 -> Switch29/1
  From374/1 -> Minus7/1
  From368/1 -> Minus3/1
  From370/1 -> Detect Decrease/1
  From376/1 -> Switch30/3
  From377/1 -> Minus5/2
  Detect Decrease/1 -> Switch29/2
  Minus7/1 -> Switch30/1
  Switch29/1 -> Goto247/1, Unit Delay9/1
  Switch31/1 -> Minus5/1, Unit Delay10/1
  From380/1 -> Switch31/2
  From381/1 -> Minus4/1
  Initial Value9/1 -> Switch29/3
  Minus5/1 -> Goto250/1
  Unit Delay10/1 -> Initial Value10/2
  From367/1 -> Initial Value10/1
  From373/1 -> Minus6/1
  Detect Increase5/1 -> Switch30/2
  Delay2/1 -> Goto249/1
  From372/1 -> Minus6/2
  From375/1 -> Detect Increase5/1
  Switch30/1 -> Delay2/1, Goto248/1
  Initial Value10/1 -> Switch31/3
  From357/1 -> Initial Value9/1
  Minus6/1 -> Minus7/2
  Minus3/1 -> Switch28/3
